simulink model "OR_10s_70l"  (R2023b)
(part 2 of 3)

      |     if contains(extractAfter(blocks{k,1}, '/'), 'Source')
      |         set_param(blocks{k}, 'BackgroundColor', '[0.929000, 0.490000, 0.439000]');
      |     end
      | end
      settings: NameChangeFcn=|
      | Component_Name = get_param(gcb, 'Name');
      | old_ID = get_param(gcb, 'Bus_ID');
      | 
      | pattern = '_\d+';
      | match = regexp(Component_Name, pattern, 'match');
      | 
      | if ~isempty(match)
      |     if ~isequal(old_ID, num2str(strtrim(extractAfter(Component_Name, '_'))))
      |         set_param(gcb, 'Bus_ID', num2str(strtrim(extractAfter(Component_Name, '_'))));
      |     end
      | else
      |     newName = [Component_Name '_' old_ID];
      |     set_param(gcb, 'Name', newName);
      | end
      | 
      | if ~isequal(old_ID, get_param(gcb, 'Bus_ID'))
      | 
      |     data = get_param(gcb, 'PortConnectivity');
      |     for i = 1:numel(data)
      |         sourceHandle = data(i,1).SrcBlock;
      |         if ~isempty(sourceHandle) && sourceHandle ~= -1
      |             sourceParams = get_param(sourceHandle, 'DialogParameters');
      |             fn = fieldnames(sourceParams);
      |             if contains(fn{2}, 'Source')
      |                 Bus_ID = get_param(gcb, 'Bus_ID');
      |                 set_param(sourceHandle, 'Source_ID', Bus_ID);
      |             end
      |         end
      |     end
      | 
      |     blocks = find_system(gcs, 'SearchDepth', 1, 'Type', 'Block');
      | 
      |     for k = 1:length(blocks)
      |         if contains(extractAfter(blocks{k,1}, '/'), 'Source')
      |             set_param(blocks{k}, 'BackgroundColor', '[0.929000, 0.490000, 0.439000]');
      |         end
      |     end
      | 
      | end
      settings: PreDeleteFcn=|
      | blocks = find_system(gcs, 'SearchDepth', 1, 'Type', 'Block');
      | 
      | for k = 1:length(blocks)
      |     if contains(extractAfter(blocks{k,1}, '/'), 'Source')
      |         set_param(blocks{k}, 'BackgroundColor', '[0.929000, 0.490000, 0.439000]');
      |     end
      | end
  Bus_60 : MATLAB Function  TreatAsAtomicUnit=on  mask{MyInitialization=0, Bus_ID=60, Fault_flag=1}
      mask prompts: Bus_ID "Bus ID"; Fault_flag "Fault flag"
      settings: CopyFcn=|
      | Component_Name = get_param(gcb, 'Name');
      | set_param(gcb, 'Bus_ID', num2str(strtrim(extractAfter(Component_Name, '_'))));
      | 
      | blocks = find_system(gcs, 'SearchDepth', 1, 'Type', 'Block');
      | 
      | for k = 1:length(blocks)
      |     if contains(extractAfter(blocks{k,1}, '/'), 'Source')
      |         set_param(blocks{k}, 'BackgroundColor', '[0.929000, 0.490000, 0.439000]');
      |     end
      | end
      settings: NameChangeFcn=|
      | Component_Name = get_param(gcb, 'Name');
      | old_ID = get_param(gcb, 'Bus_ID');
      | 
      | pattern = '_\d+';
      | match = regexp(Component_Name, pattern, 'match');
      | 
      | if ~isempty(match)
      |     if ~isequal(old_ID, num2str(strtrim(extractAfter(Component_Name, '_'))))
      |         set_param(gcb, 'Bus_ID', num2str(strtrim(extractAfter(Component_Name, '_'))));
      |     end
      | else
      |     newName = [Component_Name '_' old_ID];
      |     set_param(gcb, 'Name', newName);
      | end
      | 
      | if ~isequal(old_ID, get_param(gcb, 'Bus_ID'))
      | 
      |     data = get_param(gcb, 'PortConnectivity');
      |     for i = 1:numel(data)
      |         sourceHandle = data(i,1).SrcBlock;
      |         if ~isempty(sourceHandle) && sourceHandle ~= -1
      |             sourceParams = get_param(sourceHandle, 'DialogParameters');
      |             fn = fieldnames(sourceParams);
      |             if contains(fn{2}, 'Source')
      |                 Bus_ID = get_param(gcb, 'Bus_ID');
      |                 set_param(sourceHandle, 'Source_ID', Bus_ID);
      |             end
      |         end
      |     end
      | 
      |     blocks = find_system(gcs, 'SearchDepth', 1, 'Type', 'Block');
      | 
      |     for k = 1:length(blocks)
      |         if contains(extractAfter(blocks{k,1}, '/'), 'Source')
      |             set_param(blocks{k}, 'BackgroundColor', '[0.929000, 0.490000, 0.439000]');
      |         end
      |     end
      | 
      | end
      settings: PreDeleteFcn=|
      | blocks = find_system(gcs, 'SearchDepth', 1, 'Type', 'Block');
      | 
      | for k = 1:length(blocks)
      |     if contains(extractAfter(blocks{k,1}, '/'), 'Source')
      |         set_param(blocks{k}, 'BackgroundColor', '[0.929000, 0.490000, 0.439000]');
      |     end
      | end
  Bus_61 : MATLAB Function  TreatAsAtomicUnit=on  mask{MyInitialization=0, Bus_ID=61, Fault_flag=1}
      mask prompts: Bus_ID "Bus ID"; Fault_flag "Fault flag"
      settings: CopyFcn=|
      | Component_Name = get_param(gcb, 'Name');
      | set_param(gcb, 'Bus_ID', num2str(strtrim(extractAfter(Component_Name, '_'))));
      | 
      | blocks = find_system(gcs, 'SearchDepth', 1, 'Type', 'Block');
      | 
      | for k = 1:length(blocks)
      |     if contains(extractAfter(blocks{k,1}, '/'), 'Source')
      |         set_param(blocks{k}, 'BackgroundColor', '[0.929000, 0.490000, 0.439000]');
      |     end
      | end
      settings: NameChangeFcn=|
      | Component_Name = get_param(gcb, 'Name');
      | old_ID = get_param(gcb, 'Bus_ID');
      | 
      | pattern = '_\d+';
      | match = regexp(Component_Name, pattern, 'match');
      | 
      | if ~isempty(match)
      |     if ~isequal(old_ID, num2str(strtrim(extractAfter(Component_Name, '_'))))
      |         set_param(gcb, 'Bus_ID', num2str(strtrim(extractAfter(Component_Name, '_'))));
      |     end
      | else
      |     newName = [Component_Name '_' old_ID];
      |     set_param(gcb, 'Name', newName);
      | end
      | 
      | if ~isequal(old_ID, get_param(gcb, 'Bus_ID'))
      | 
      |     data = get_param(gcb, 'PortConnectivity');
      |     for i = 1:numel(data)
      |         sourceHandle = data(i,1).SrcBlock;
      |         if ~isempty(sourceHandle) && sourceHandle ~= -1
      |             sourceParams = get_param(sourceHandle, 'DialogParameters');
      |             fn = fieldnames(sourceParams);
      |             if contains(fn{2}, 'Source')
      |                 Bus_ID = get_param(gcb, 'Bus_ID');
      |                 set_param(sourceHandle, 'Source_ID', Bus_ID);
      |             end
      |         end
      |     end
      | 
      |     blocks = find_system(gcs, 'SearchDepth', 1, 'Type', 'Block');
      | 
      |     for k = 1:length(blocks)
      |         if contains(extractAfter(blocks{k,1}, '/'), 'Source')
      |             set_param(blocks{k}, 'BackgroundColor', '[0.929000, 0.490000, 0.439000]');
      |         end
      |     end
      | 
      | end
      settings: PreDeleteFcn=|
      | blocks = find_system(gcs, 'SearchDepth', 1, 'Type', 'Block');
      | 
      | for k = 1:length(blocks)
      |     if contains(extractAfter(blocks{k,1}, '/'), 'Source')
      |         set_param(blocks{k}, 'BackgroundColor', '[0.929000, 0.490000, 0.439000]');
      |     end
      | end
  Bus_62 : MATLAB Function  TreatAsAtomicUnit=on  mask{MyInitialization=0, Bus_ID=62, Fault_flag=1}
      mask prompts: Bus_ID "Bus ID"; Fault_flag "Fault flag"
      settings: CopyFcn=|
      | Component_Name = get_param(gcb, 'Name');
      | set_param(gcb, 'Bus_ID', num2str(strtrim(extractAfter(Component_Name, '_'))));
      | 
      | blocks = find_system(gcs, 'SearchDepth', 1, 'Type', 'Block');
      | 
      | for k = 1:length(blocks)
      |     if contains(extractAfter(blocks{k,1}, '/'), 'Source')
      |         set_param(blocks{k}, 'BackgroundColor', '[0.929000, 0.490000, 0.439000]');
      |     end
      | end
      settings: NameChangeFcn=|
      | Component_Name = get_param(gcb, 'Name');
      | old_ID = get_param(gcb, 'Bus_ID');
      | 
      | pattern = '_\d+';
      | match = regexp(Component_Name, pattern, 'match');
      | 
      | if ~isempty(match)
      |     if ~isequal(old_ID, num2str(strtrim(extractAfter(Component_Name, '_'))))
      |         set_param(gcb, 'Bus_ID', num2str(strtrim(extractAfter(Component_Name, '_'))));
      |     end
      | else
      |     newName = [Component_Name '_' old_ID];
      |     set_param(gcb, 'Name', newName);
      | end
      | 
      | if ~isequal(old_ID, get_param(gcb, 'Bus_ID'))
      | 
      |     data = get_param(gcb, 'PortConnectivity');
      |     for i = 1:numel(data)
      |         sourceHandle = data(i,1).SrcBlock;
      |         if ~isempty(sourceHandle) && sourceHandle ~= -1
      |             sourceParams = get_param(sourceHandle, 'DialogParameters');
      |             fn = fieldnames(sourceParams);
      |             if contains(fn{2}, 'Source')
      |                 Bus_ID = get_param(gcb, 'Bus_ID');
      |                 set_param(sourceHandle, 'Source_ID', Bus_ID);
      |             end
      |         end
      |     end
      | 
      |     blocks = find_system(gcs, 'SearchDepth', 1, 'Type', 'Block');
      | 
      |     for k = 1:length(blocks)
      |         if contains(extractAfter(blocks{k,1}, '/'), 'Source')
      |             set_param(blocks{k}, 'BackgroundColor', '[0.929000, 0.490000, 0.439000]');
      |         end
      |     end
      | 
      | end
      settings: PreDeleteFcn=|
      | blocks = find_system(gcs, 'SearchDepth', 1, 'Type', 'Block');
      | 
      | for k = 1:length(blocks)
      |     if contains(extractAfter(blocks{k,1}, '/'), 'Source')
      |         set_param(blocks{k}, 'BackgroundColor', '[0.929000, 0.490000, 0.439000]');
      |     end
      | end
  Bus_63 : MATLAB Function  TreatAsAtomicUnit=on  mask{MyInitialization=0, Bus_ID=63, Fault_flag=1}
      mask prompts: Bus_ID "Bus ID"; Fault_flag "Fault flag"
      settings: CopyFcn=|
      | Component_Name = get_param(gcb, 'Name');
      | set_param(gcb, 'Bus_ID', num2str(strtrim(extractAfter(Component_Name, '_'))));
      | 
      | blocks = find_system(gcs, 'SearchDepth', 1, 'Type', 'Block');
      | 
      | for k = 1:length(blocks)
      |     if contains(extractAfter(blocks{k,1}, '/'), 'Source')
      |         set_param(blocks{k}, 'BackgroundColor', '[0.929000, 0.490000, 0.439000]');
      |     end
      | end
      settings: NameChangeFcn=|
      | Component_Name = get_param(gcb, 'Name');
      | old_ID = get_param(gcb, 'Bus_ID');
      | 
      | pattern = '_\d+';
      | match = regexp(Component_Name, pattern, 'match');
      | 
      | if ~isempty(match)
      |     if ~isequal(old_ID, num2str(strtrim(extractAfter(Component_Name, '_'))))
      |         set_param(gcb, 'Bus_ID', num2str(strtrim(extractAfter(Component_Name, '_'))));
      |     end
      | else
      |     newName = [Component_Name '_' old_ID];
      |     set_param(gcb, 'Name', newName);
      | end
      | 
      | if ~isequal(old_ID, get_param(gcb, 'Bus_ID'))
      | 
      |     data = get_param(gcb, 'PortConnectivity');
      |     for i = 1:numel(data)
      |         sourceHandle = data(i,1).SrcBlock;
      |         if ~isempty(sourceHandle) && sourceHandle ~= -1
      |             sourceParams = get_param(sourceHandle, 'DialogParameters');
      |             fn = fieldnames(sourceParams);
      |             if contains(fn{2}, 'Source')
      |                 Bus_ID = get_param(gcb, 'Bus_ID');
      |                 set_param(sourceHandle, 'Source_ID', Bus_ID);
      |             end
      |         end
      |     end
      | 
      |     blocks = find_system(gcs, 'SearchDepth', 1, 'Type', 'Block');
      | 
      |     for k = 1:length(blocks)
      |         if contains(extractAfter(blocks{k,1}, '/'), 'Source')
      |             set_param(blocks{k}, 'BackgroundColor', '[0.929000, 0.490000, 0.439000]');
      |         end
      |     end
      | 
      | end
      settings: PreDeleteFcn=|
      | blocks = find_system(gcs, 'SearchDepth', 1, 'Type', 'Block');
      | 
      | for k = 1:length(blocks)
      |     if contains(extractAfter(blocks{k,1}, '/'), 'Source')
      |         set_param(blocks{k}, 'BackgroundColor', '[0.929000, 0.490000, 0.439000]');
      |     end
      | end
  Bus_64 : MATLAB Function  TreatAsAtomicUnit=on  mask{MyInitialization=0, Bus_ID=64, Fault_flag=1}
      mask prompts: Bus_ID "Bus ID"; Fault_flag "Fault flag"
      settings: CopyFcn=|
      | Component_Name = get_param(gcb, 'Name');
      | set_param(gcb, 'Bus_ID', num2str(strtrim(extractAfter(Component_Name, '_'))));
      | 
      | blocks = find_system(gcs, 'SearchDepth', 1, 'Type', 'Block');
      | 
      | for k = 1:length(blocks)
      |     if contains(extractAfter(blocks{k,1}, '/'), 'Source')
      |         set_param(blocks{k}, 'BackgroundColor', '[0.929000, 0.490000, 0.439000]');
      |     end
      | end
      settings: NameChangeFcn=|
      | Component_Name = get_param(gcb, 'Name');
      | old_ID = get_param(gcb, 'Bus_ID');
      | 
      | pattern = '_\d+';
      | match = regexp(Component_Name, pattern, 'match');
      | 
      | if ~isempty(match)
      |     if ~isequal(old_ID, num2str(strtrim(extractAfter(Component_Name, '_'))))
      |         set_param(gcb, 'Bus_ID', num2str(strtrim(extractAfter(Component_Name, '_'))));
      |     end
      | else
      |     newName = [Component_Name '_' old_ID];
      |     set_param(gcb, 'Name', newName);
      | end
      | 
      | if ~isequal(old_ID, get_param(gcb, 'Bus_ID'))
      | 
      |     data = get_param(gcb, 'PortConnectivity');
      |     for i = 1:numel(data)
      |         sourceHandle = data(i,1).SrcBlock;
      |         if ~isempty(sourceHandle) && sourceHandle ~= -1
      |             sourceParams = get_param(sourceHandle, 'DialogParameters');
      |             fn = fieldnames(sourceParams);
      |             if contains(fn{2}, 'Source')
      |                 Bus_ID = get_param(gcb, 'Bus_ID');
      |                 set_param(sourceHandle, 'Source_ID', Bus_ID);
      |             end
      |         end
      |     end
      | 
      |     blocks = find_system(gcs, 'SearchDepth', 1, 'Type', 'Block');
      | 
      |     for k = 1:length(blocks)
      |         if contains(extractAfter(blocks{k,1}, '/'), 'Source')
      |             set_param(blocks{k}, 'BackgroundColor', '[0.929000, 0.490000, 0.439000]');
      |         end
      |     end
      | 
      | end
      settings: PreDeleteFcn=|
      | blocks = find_system(gcs, 'SearchDepth', 1, 'Type', 'Block');
      | 
      | for k = 1:length(blocks)
      |     if contains(extractAfter(blocks{k,1}, '/'), 'Source')
      |         set_param(blocks{k}, 'BackgroundColor', '[0.929000, 0.490000, 0.439000]');
      |     end
      | end
  Bus_65 : MATLAB Function  TreatAsAtomicUnit=on  mask{MyInitialization=0, Bus_ID=65, Fault_flag=1}
      mask prompts: Bus_ID "Bus ID"; Fault_flag "Fault flag"
      settings: CopyFcn=|
      | Component_Name = get_param(gcb, 'Name');
      | set_param(gcb, 'Bus_ID', num2str(strtrim(extractAfter(Component_Name, '_'))));
      | 
      | blocks = find_system(gcs, 'SearchDepth', 1, 'Type', 'Block');
      | 
      | for k = 1:length(blocks)
      |     if contains(extractAfter(blocks{k,1}, '/'), 'Source')
      |         set_param(blocks{k}, 'BackgroundColor', '[0.929000, 0.490000, 0.439000]');
      |     end
      | end
      settings: NameChangeFcn=|
      | Component_Name = get_param(gcb, 'Name');
      | old_ID = get_param(gcb, 'Bus_ID');
      | 
      | pattern = '_\d+';
      | match = regexp(Component_Name, pattern, 'match');
      | 
      | if ~isempty(match)
      |     if ~isequal(old_ID, num2str(strtrim(extractAfter(Component_Name, '_'))))
      |         set_param(gcb, 'Bus_ID', num2str(strtrim(extractAfter(Component_Name, '_'))));
      |     end
      | else
      |     newName = [Component_Name '_' old_ID];
      |     set_param(gcb, 'Name', newName);
      | end
      | 
      | if ~isequal(old_ID, get_param(gcb, 'Bus_ID'))
      | 
      |     data = get_param(gcb, 'PortConnectivity');
      |     for i = 1:numel(data)
      |         sourceHandle = data(i,1).SrcBlock;
      |         if ~isempty(sourceHandle) && sourceHandle ~= -1
      |             sourceParams = get_param(sourceHandle, 'DialogParameters');
      |             fn = fieldnames(sourceParams);
      |             if contains(fn{2}, 'Source')
      |                 Bus_ID = get_param(gcb, 'Bus_ID');
      |                 set_param(sourceHandle, 'Source_ID', Bus_ID);
      |             end
      |         end
      |     end
      | 
      |     blocks = find_system(gcs, 'SearchDepth', 1, 'Type', 'Block');
      | 
      |     for k = 1:length(blocks)
      |         if contains(extractAfter(blocks{k,1}, '/'), 'Source')
      |             set_param(blocks{k}, 'BackgroundColor', '[0.929000, 0.490000, 0.439000]');
      |         end
      |     end
      | 
      | end
      settings: PreDeleteFcn=|
      | blocks = find_system(gcs, 'SearchDepth', 1, 'Type', 'Block');
      | 
      | for k = 1:length(blocks)
      |     if contains(extractAfter(blocks{k,1}, '/'), 'Source')
      |         set_param(blocks{k}, 'BackgroundColor', '[0.929000, 0.490000, 0.439000]');
      |     end
      | end
  Bus_7 : MATLAB Function  TreatAsAtomicUnit=on  mask{MyInitialization=0, Bus_ID=7, Fault_flag=1}
      mask prompts: Bus_ID "Bus ID"; Fault_flag "Fault flag"
      settings: CopyFcn=|
      | Component_Name = get_param(gcb, 'Name');
      | set_param(gcb, 'Bus_ID', num2str(strtrim(extractAfter(Component_Name, '_'))));
      | 
      | blocks = find_system(gcs, 'SearchDepth', 1, 'Type', 'Block');
      | 
      | for k = 1:length(blocks)
      |     if contains(extractAfter(blocks{k,1}, '/'), 'Source')
      |         set_param(blocks{k}, 'BackgroundColor', '[0.929000, 0.490000, 0.439000]');
      |     end
      | end
      settings: NameChangeFcn=|
      | Component_Name = get_param(gcb, 'Name');
      | old_ID = get_param(gcb, 'Bus_ID');
      | 
      | pattern = '_\d+';
      | match = regexp(Component_Name, pattern, 'match');
      | 
      | if ~isempty(match)
      |     if ~isequal(old_ID, num2str(strtrim(extractAfter(Component_Name, '_'))))
      |         set_param(gcb, 'Bus_ID', num2str(strtrim(extractAfter(Component_Name, '_'))));
      |     end
      | else
      |     newName = [Component_Name '_' old_ID];
      |     set_param(gcb, 'Name', newName);
      | end
      | 
      | if ~isequal(old_ID, get_param(gcb, 'Bus_ID'))
      | 
      |     data = get_param(gcb, 'PortConnectivity');
      |     for i = 1:numel(data)
      |         sourceHandle = data(i,1).SrcBlock;
      |         if ~isempty(sourceHandle) && sourceHandle ~= -1
      |             sourceParams = get_param(sourceHandle, 'DialogParameters');
      |             fn = fieldnames(sourceParams);
      |             if contains(fn{2}, 'Source')
      |                 Bus_ID = get_param(gcb, 'Bus_ID');
      |                 set_param(sourceHandle, 'Source_ID', Bus_ID);
      |             end
      |         end
      |     end
      | 
      |     blocks = find_system(gcs, 'SearchDepth', 1, 'Type', 'Block');
      | 
      |     for k = 1:length(blocks)
      |         if contains(extractAfter(blocks{k,1}, '/'), 'Source')
      |             set_param(blocks{k}, 'BackgroundColor', '[0.929000, 0.490000, 0.439000]');
      |         end
      |     end
      | 
      | end
      settings: PreDeleteFcn=|
      | blocks = find_system(gcs, 'SearchDepth', 1, 'Type', 'Block');
      | 
      | for k = 1:length(blocks)
      |     if contains(extractAfter(blocks{k,1}, '/'), 'Source')
      |         set_param(blocks{k}, 'BackgroundColor', '[0.929000, 0.490000, 0.439000]');
      |     end
      | end
  Bus_8 : MATLAB Function  TreatAsAtomicUnit=on  mask{MyInitialization=0, Bus_ID=8, Fault_flag=0}
      mask prompts: Bus_ID "Bus ID"; Fault_flag "Fault flag"
      settings: CopyFcn=|
      | Component_Name = get_param(gcb, 'Name');
      | set_param(gcb, 'Bus_ID', num2str(strtrim(extractAfter(Component_Name, '_'))));
      | 
      | blocks = find_system(gcs, 'SearchDepth', 1, 'Type', 'Block');
      | 
      | for k = 1:length(blocks)
      |     if contains(extractAfter(blocks{k,1}, '/'), 'Source')
      |         set_param(blocks{k}, 'BackgroundColor', '[0.929000, 0.490000, 0.439000]');
      |     end
      | end
      settings: NameChangeFcn=|
      | Component_Name = get_param(gcb, 'Name');
      | old_ID = get_param(gcb, 'Bus_ID');
      | 
      | pattern = '_\d+';
      | match = regexp(Component_Name, pattern, 'match');
      | 
      | if ~isempty(match)
      |     if ~isequal(old_ID, num2str(strtrim(extractAfter(Component_Name, '_'))))
      |         set_param(gcb, 'Bus_ID', num2str(strtrim(extractAfter(Component_Name, '_'))));
      |     end
      | else
      |     newName = [Component_Name '_' old_ID];
      |     set_param(gcb, 'Name', newName);
      | end
      | 
      | if ~isequal(old_ID, get_param(gcb, 'Bus_ID'))
      | 
      |     data = get_param(gcb, 'PortConnectivity');
      |     for i = 1:numel(data)
      |         sourceHandle = data(i,1).SrcBlock;
      |         if ~isempty(sourceHandle) && sourceHandle ~= -1
      |             sourceParams = get_param(sourceHandle, 'DialogParameters');
      |             fn = fieldnames(sourceParams);
      |             if contains(fn{2}, 'Source')
      |                 Bus_ID = get_param(gcb, 'Bus_ID');
      |                 set_param(sourceHandle, 'Source_ID', Bus_ID);
      |             end
      |         end
      |     end
      | 
      |     blocks = find_system(gcs, 'SearchDepth', 1, 'Type', 'Block');
      | 
      |     for k = 1:length(blocks)
      |         if contains(extractAfter(blocks{k,1}, '/'), 'Source')
      |             set_param(blocks{k}, 'BackgroundColor', '[0.929000, 0.490000, 0.439000]');
      |         end
      |     end
      | 
      | end
      settings: PreDeleteFcn=|
      | blocks = find_system(gcs, 'SearchDepth', 1, 'Type', 'Block');
      | 
      | for k = 1:length(blocks)
      |     if contains(extractAfter(blocks{k,1}, '/'), 'Source')
      |         set_param(blocks{k}, 'BackgroundColor', '[0.929000, 0.490000, 0.439000]');
      |     end
      | end
  Bus_9 : MATLAB Function  TreatAsAtomicUnit=on  mask{MyInitialization=0, Bus_ID=9, Fault_flag=1}
      mask prompts: Bus_ID "Bus ID"; Fault_flag "Fault flag"
      settings: CopyFcn=|
      | Component_Name = get_param(gcb, 'Name');
      | set_param(gcb, 'Bus_ID', num2str(strtrim(extractAfter(Component_Name, '_'))));
      | 
      | blocks = find_system(gcs, 'SearchDepth', 1, 'Type', 'Block');
      | 
      | for k = 1:length(blocks)
      |     if contains(extractAfter(blocks{k,1}, '/'), 'Source')
      |         set_param(blocks{k}, 'BackgroundColor', '[0.929000, 0.490000, 0.439000]');
      |     end
      | end
      settings: NameChangeFcn=|
      | Component_Name = get_param(gcb, 'Name');
      | old_ID = get_param(gcb, 'Bus_ID');
      | 
      | pattern = '_\d+';
      | match = regexp(Component_Name, pattern, 'match');
      | 
      | if ~isempty(match)
      |     if ~isequal(old_ID, num2str(strtrim(extractAfter(Component_Name, '_'))))
      |         set_param(gcb, 'Bus_ID', num2str(strtrim(extractAfter(Component_Name, '_'))));
      |     end
      | else
      |     newName = [Component_Name '_' old_ID];
      |     set_param(gcb, 'Name', newName);
      | end
      | 
      | if ~isequal(old_ID, get_param(gcb, 'Bus_ID'))
      | 
      |     data = get_param(gcb, 'PortConnectivity');
      |     for i = 1:numel(data)
      |         sourceHandle = data(i,1).SrcBlock;
      |         if ~isempty(sourceHandle) && sourceHandle ~= -1
      |             sourceParams = get_param(sourceHandle, 'DialogParameters');
      |             fn = fieldnames(sourceParams);
      |             if contains(fn{2}, 'Source')
      |                 Bus_ID = get_param(gcb, 'Bus_ID');
      |                 set_param(sourceHandle, 'Source_ID', Bus_ID);
      |             end
      |         end
      |     end
      | 
      |     blocks = find_system(gcs, 'SearchDepth', 1, 'Type', 'Block');
      | 
      |     for k = 1:length(blocks)
      |         if contains(extractAfter(blocks{k,1}, '/'), 'Source')
      |             set_param(blocks{k}, 'BackgroundColor', '[0.929000, 0.490000, 0.439000]');
      |         end
      |     end
      | 
      | end
      settings: PreDeleteFcn=|
      | blocks = find_system(gcs, 'SearchDepth', 1, 'Type', 'Block');
      | 
      | for k = 1:length(blocks)
      |     if contains(extractAfter(blocks{k,1}, '/'), 'Source')
      |         set_param(blocks{k}, 'BackgroundColor', '[0.929000, 0.490000, 0.439000]');
      |     end
      | end
  CB_1 : ABB_UPPAAL_Library/CB_1  MyInitialization=0  CB_ID=1  Sel_Type=3  m=3  i1=900  t1=180  i2_flag=off  i2=null  t2=null  i3_flag=off  i3=null  t3=null  i7=1800  t7FW=8  t7BW=8  tselFW=1  tselBW=1  Actors={ '3', '1', '1' }
      settings: SourceProductName=ABB UPPAAL Library
  CB_10 : ABB_UPPAAL_Library/CB_1  MyInitialization=0  CB_ID=10  Sel_Type=1  m=3  i1=90  t1=160  i2_flag=on  i2=180  t2=6  i3_flag=off  i3=null  t3=null  i7=null  t7FW=null  t7BW=null  tselFW=null  tselBW=null  Actors={}
      settings: SourceProductName=ABB UPPAAL Library
  CB_11 : ABB_UPPAAL_Library/CB_1  MyInitialization=0  CB_ID=11  Sel_Type=1  m=3  i1=30  t1=100  i2_flag=on  i2=60  t2=2  i3_flag=off  i3=null  t3=null  i7=null  t7FW=null  t7BW=null  tselFW=null  tselBW=null  Actors={}
      settings: SourceProductName=ABB UPPAAL Library
  CB_12 : ABB_UPPAAL_Library/CB_1  MyInitialization=0  CB_ID=12  Sel_Type=1  m=3  i1=60  t1=120  i2_flag=on  i2=120  t2=4  i3_flag=off  i3=null  t3=null  i7=null  t7FW=null  t7BW=null  tselFW=null  tselBW=null  Actors={}
      settings: SourceProductName=ABB UPPAAL Library
  CB_13 : ABB_UPPAAL_Library/CB_1  MyInitialization=0  CB_ID=13  Sel_Type=1  m=3  i1=30  t1=100  i2_flag=on  i2=60  t2=2  i3_flag=off  i3=null  t3=null  i7=null  t7FW=null  t7BW=null  tselFW=null  tselBW=null  Actors={}
      settings: SourceProductName=ABB UPPAAL Library
  CB_14 : ABB_UPPAAL_Library/CB_1  MyInitialization=0  CB_ID=14  Sel_Type=1  m=3  i1=30  t1=100  i2_flag=on  i2=60  t2=2  i3_flag=off  i3=null  t3=null  i7=null  t7FW=null  t7BW=null  tselFW=null  tselBW=null  Actors={}
      settings: SourceProductName=ABB UPPAAL Library
  CB_15 : ABB_UPPAAL_Library/CB_1  MyInitialization=0  CB_ID=15  Sel_Type=3  m=3  i1=720  t1=170  i2_flag=off  i2=null  t2=null  i3_flag=off  i3=null  t3=null  i7=1440  t7FW=7  t7BW=7  tselFW=1  tselBW=1  Actors={ '8', '0', '0'; '9', '0', '0'; '10', '1', '0'; '16', '0', '1'; '17', '1', '1'; '22', '1', '1' }
      settings: SourceProductName=ABB UPPAAL Library
  CB_16 : ABB_UPPAAL_Library/CB_1  MyInitialization=0  CB_ID=16  Sel_Type=3  m=3  i1=900  t1=180  i2_flag=off  i2=null  t2=null  i3_flag=off  i3=null  t3=null  i7=1800  t7FW=8  t7BW=8  tselFW=1  tselBW=1  Actors={ '15', '0', '1'; '17', '1', '1'; '22', '1', '1' }
      settings: SourceProductName=ABB UPPAAL Library
  CB_17 : ABB_UPPAAL_Library/CB_1  MyInitialization=0  CB_ID=17  Sel_Type=1  m=3  i1=90  t1=160  i2_flag=on  i2=180  t2=6  i3_flag=off  i3=null  t3=null  i7=null  t7FW=null  t7BW=null  tselFW=null  tselBW=null  Actors={}
      settings: SourceProductName=ABB UPPAAL Library
  CB_18 : ABB_UPPAAL_Library/CB_1  MyInitialization=0  CB_ID=18  Sel_Type=1  m=3  i1=30  t1=100  i2_flag=on  i2=60  t2=2  i3_flag=off  i3=null  t3=null  i7=null  t7FW=null  t7BW=null  tselFW=null  tselBW=null  Actors={}
      settings: SourceProductName=ABB UPPAAL Library
  CB_19 : ABB_UPPAAL_Library/CB_1  MyInitialization=0  CB_ID=19  Sel_Type=1  m=3  i1=30  t1=100  i2_flag=on  i2=60  t2=2  i3_flag=off  i3=null  t3=null  i7=null  t7FW=null  t7BW=null  tselFW=null  tselBW=null  Actors={}
      settings: SourceProductName=ABB UPPAAL Library
  CB_2 : ABB_UPPAAL_Library/CB_1  MyInitialization=0  CB_ID=2  Sel_Type=3  m=3  i1=900  t1=180  i2_flag=off  i2=null  t2=null  i3_flag=off  i3=null  t3=null  i7=1800  t7FW=8  t7BW=8  tselFW=1  tselBW=1  Actors={ '3', '0', '1'; '4', '1', '1'; '9', '1', '1' }
      settings: SourceProductName=ABB UPPAAL Library
  CB_20 : ABB_UPPAAL_Library/CB_1  MyInitialization=0  CB_ID=20  Sel_Type=1  m=3  i1=30  t1=100  i2_flag=on  i2=60  t2=2  i3_flag=off  i3=null  t3=null  i7=null  t7FW=null  t7BW=null  tselFW=null  tselBW=null  Actors={}
      settings: SourceProductName=ABB UPPAAL Library
  CB_21 : ABB_UPPAAL_Library/CB_1  MyInitialization=0  CB_ID=21  Sel_Type=3  m=3  i1=900  t1=180  i2_flag=off  i2=null  t2=null  i3_flag=off  i3=null  t3=null  i7=1800  t7FW=8  t7BW=8  tselFW=1  tselBW=1  Actors={ '22', '0', '1'; '30', '1', '1'; '31', '1', '1' }
      settings: SourceProductName=ABB UPPAAL Library
  CB_22 : ABB_UPPAAL_Library/CB_1  MyInitialization=0  CB_ID=22  Sel_Type=3  m=3  i1=630  t1=170  i2_flag=off  i2=null  t2=null  i3_flag=off  i3=null  t3=null  i7=1260  t7FW=7  t7BW=7  tselFW=1  tselBW=1  Actors={ '15', '0', '0'; '16', '0', '0'; '17', '1', '0'; '21', '0', '1'; '30', '1', '1'; '31', '1', '1' }
      settings: SourceProductName=ABB UPPAAL Library
  CB_23 : ABB_UPPAAL_Library/CB_1  MyInitialization=0  CB_ID=23  Sel_Type=1  m=3  i1=90  t1=160  i2_flag=on  i2=180  t2=6  i3_flag=off  i3=null  t3=null  i7=null  t7FW=null  t7BW=null  tselFW=null  tselBW=null  Actors={}
      settings: SourceProductName=ABB UPPAAL Library
  CB_24 : ABB_UPPAAL_Library/CB_1  MyInitialization=0  CB_ID=24  Sel_Type=1  m=3  i1=30  t1=100  i2_flag=on  i2=60  t2=2  i3_flag=off  i3=null  t3=null  i7=null  t7FW=null  t7BW=null  tselFW=null  tselBW=null  Actors={}
      settings: SourceProductName=ABB UPPAAL Library
  CB_25 : ABB_UPPAAL_Library/CB_1  MyInitialization=0  CB_ID=25  Sel_Type=1  m=3  i1=60  t1=120  i2_flag=on  i2=120  t2=4  i3_flag=off  i3=null  t3=null  i7=null  t7FW=null  t7BW=null  tselFW=null  tselBW=null  Actors={}
      settings: SourceProductName=ABB UPPAAL Library
  CB_26 : ABB_UPPAAL_Library/CB_1  MyInitialization=0  CB_ID=26  Sel_Type=1  m=3  i1=30  t1=100  i2_flag=on  i2=60  t2=2  i3_flag=off  i3=null  t3=null  i7=null  t7FW=null  t7BW=null  tselFW=null  tselBW=null  Actors={}
      settings: SourceProductName=ABB UPPAAL Library
  CB_27 : ABB_UPPAAL_Library/CB_1  MyInitialization=0  CB_ID=27  Sel_Type=1  m=3  i1=30  t1=100  i2_flag=on  i2=60  t2=2  i3_flag=off  i3=null  t3=null  i7=null  t7FW=null  t7BW=null  tselFW=null  tselBW=null  Actors={}
      settings: SourceProductName=ABB UPPAAL Library
  CB_28 : ABB_UPPAAL_Library/CB_1  MyInitialization=0  CB_ID=28  Sel_Type=3  m=3  i1=310  t1=170  i2_flag=off  i2=null  t2=null  i3_flag=off  i3=null  t3=null  i7=620  t7FW=7  t7BW=7  tselFW=1  tselBW=1  Actors={ '23', '1', '0'; '29', '0', '0'; '30', '0', '0'; '32', '1', '1'; '37', '1', '1'; '38', '0', '1' }
      settings: SourceProductName=ABB UPPAAL Library
  CB_29 : ABB_UPPAAL_Library/CB_1  MyInitialization=0  CB_ID=29  Sel_Type=3  m=3  i1=900  t1=180  i2_flag=off  i2=null  t2=null  i3_flag=off  i3=null  t3=null  i7=1800  t7FW=8  t7BW=8  tselFW=1  tselBW=1  Actors={ '23', '1', '1'; '28', '1', '1'; '30', '0', '1' }
      settings: SourceProductName=ABB UPPAAL Library
  CB_3 : ABB_UPPAAL_Library/CB_1  MyInitialization=0  CB_ID=3  Sel_Type=3  m=3  i1=900  t1=170  i2_flag=off  i2=null  t2=null  i3_flag=off  i3=null  t3=null  i7=1800  t7FW=7  t7BW=7  tselFW=1  tselBW=1  Actors={ '1', '0', '0'; '2', '0', '1'; '4', '1', '1'; '9', '1', '1' }
      settings: SourceProductName=ABB UPPAAL Library
  CB_30 : ABB_UPPAAL_Library/CB_1  MyInitialization=0  CB_ID=30  Sel_Type=3  m=3  i1=600  t1=170  i2_flag=off  i2=null  t2=null  i3_flag=off  i3=null  t3=null  i7=1200  t7FW=7  t7BW=7  tselFW=1  tselBW=1  Actors={ '21', '0', '0'; '22', '0', '0'; '23', '1', '1'; '28', '1', '1'; '29', '0', '1'; '31', '1', '0' }
      settings: SourceProductName=ABB UPPAAL Library
  CB_31 : ABB_UPPAAL_Library/CB_1  MyInitialization=0  CB_ID=31  Sel_Type=1  m=3  i1=30  t1=100  i2_flag=on  i2=60  t2=2  i3_flag=off  i3=null  t3=null  i7=null  t7FW=null  t7BW=null  tselFW=null  tselBW=null  Actors={}
      settings: SourceProductName=ABB UPPAAL Library
  CB_32 : ABB_UPPAAL_Library/CB_1  MyInitialization=0  CB_ID=32  Sel_Type=1  m=3  i1=90  t1=160  i2_flag=on  i2=180  t2=6  i3_flag=off  i3=null  t3=null  i7=null  t7FW=null  t7BW=null  tselFW=null  tselBW=null  Actors={}
      settings: SourceProductName=ABB UPPAAL Library
  CB_33 : ABB_UPPAAL_Library/CB_1  MyInitialization=0  CB_ID=33  Sel_Type=1  m=3  i1=30  t1=100  i2_flag=on  i2=60  t2=2  i3_flag=off  i3=null  t3=null  i7=null  t7FW=null  t7BW=null  tselFW=null  tselBW=null  Actors={}
      settings: SourceProductName=ABB UPPAAL Library
  CB_34 : ABB_UPPAAL_Library/CB_1  MyInitialization=0  CB_ID=34  Sel_Type=1  m=3  i1=60  t1=120  i2_flag=on  i2=120  t2=4  i3_flag=off  i3=null  t3=null  i7=null  t7FW=null  t7BW=null  tselFW=null  tselBW=null  Actors={}
      settings: SourceProductName=ABB UPPAAL Library
  CB_35 : ABB_UPPAAL_Library/CB_1  MyInitialization=0  CB_ID=35  Sel_Type=1  m=3  i1=30  t1=100  i2_flag=on  i2=60  t2=2  i3_flag=off  i3=null  t3=null  i7=null  t7FW=null  t7BW=null  tselFW=null  tselBW=null  Actors={}
      settings: SourceProductName=ABB UPPAAL Library
  CB_36 : ABB_UPPAAL_Library/CB_1  MyInitialization=0  CB_ID=36  Sel_Type=1  m=3  i1=30  t1=100  i2_flag=on  i2=60  t2=2  i3_flag=off  i3=null  t3=null  i7=null  t7FW=null  t7BW=null  tselFW=null  tselBW=null  Actors={}
      settings: SourceProductName=ABB UPPAAL Library
  CB_37 : ABB_UPPAAL_Library/CB_1  MyInitialization=0  CB_ID=37  Sel_Type=3  m=3  i1=480  t1=170  i2_flag=off  i2=null  t2=null  i3_flag=off  i3=null  t3=null  i7=960  t7FW=7  t7BW=7  tselFW=1  tselBW=1  Actors={ '28', '0', '0'; '32', '1', '0'; '38', '0', '0'; '39', '1', '1'; '44', '1', '1'; '45', '0', '1' }
      settings: SourceProductName=ABB UPPAAL Library
  CB_38 : ABB_UPPAAL_Library/CB_1  MyInitialization=0  CB_ID=38  Sel_Type=3  m=3  i1=900  t1=180  i2_flag=off  i2=null  t2=null  i3_flag=off  i3=null  t3=null  i7=1800  t7FW=8  t7BW=8  tselFW=1  tselBW=1  Actors={ '28', '0', '1'; '32', '1', '1'; '37', '1', '1' }
      settings: SourceProductName=ABB UPPAAL Library
  CB_39 : ABB_UPPAAL_Library/CB_1  MyInitialization=0  CB_ID=39  Sel_Type=1  m=3  i1=90  t1=160  i2_flag=on  i2=180  t2=6  i3_flag=off  i3=null  t3=null  i7=null  t7FW=null  t7BW=null  tselFW=null  tselBW=null  Actors={}
      settings: SourceProductName=ABB UPPAAL Library
  CB_4 : ABB_UPPAAL_Library/CB_1  MyInitialization=0  CB_ID=4  Sel_Type=1  m=3  i1=90  t1=120  i2_flag=on  i2=180  t2=4  i3_flag=off  i3=null  t3=null  i7=null  t7FW=null  t7BW=null  tselFW=null  tselBW=null  Actors={}
      settings: SourceProductName=ABB UPPAAL Library
  CB_40 : ABB_UPPAAL_Library/CB_1  MyInitialization=0  CB_ID=40  Sel_Type=1  m=3  i1=30  t1=100  i2_flag=on  i2=60  t2=2  i3_flag=off  i3=null  t3=null  i7=null  t7FW=null  t7BW=null  tselFW=null  tselBW=null  Actors={}
      settings: SourceProductName=ABB UPPAAL Library
  CB_41 : ABB_UPPAAL_Library/CB_1  MyInitialization=0  CB_ID=41  Sel_Type=1  m=3  i1=60  t1=120  i2_flag=on  i2=120  t2=4  i3_flag=off  i3=null  t3=null  i7=null  t7FW=null  t7BW=null  tselFW=null  tselBW=null  Actors={}
      settings: SourceProductName=ABB UPPAAL Library
  CB_42 : ABB_UPPAAL_Library/CB_1  MyInitialization=0  CB_ID=42  Sel_Type=1  m=3  i1=30  t1=100  i2_flag=on  i2=60  t2=2  i3_flag=off  i3=null  t3=null  i7=null  t7FW=null  t7BW=null  tselFW=null  tselBW=null  Actors={}
      settings: SourceProductName=ABB UPPAAL Library
  CB_43 : ABB_UPPAAL_Library/CB_1  MyInitialization=0  CB_ID=43  Sel_Type=1  m=3  i1=30  t1=100  i2_flag=on  i2=60  t2=2  i3_flag=off  i3=null  t3=null  i7=null  t7FW=null  t7BW=null  tselFW=null  tselBW=null  Actors={}
      settings: SourceProductName=ABB UPPAAL Library
  CB_44 : ABB_UPPAAL_Library/CB_1  MyInitialization=0  CB_ID=44  Sel_Type=3  m=3  i1=570  t1=170  i2_flag=off  i2=null  t2=null  i3_flag=off  i3=null  t3=null  i7=1140  t7FW=7  t7BW=7  tselFW=1  tselBW=1  Actors={ '37', '0', '0'; '39', '1', '0'; '45', '0', '0'; '46', '1', '1'; '51', '1', '1'; '52', '0', '1' }
      settings: SourceProductName=ABB UPPAAL Library
  CB_45 : ABB_UPPAAL_Library/CB_1  MyInitialization=0  CB_ID=45  Sel_Type=3  m=3  i1=900  t1=180  i2_flag=off  i2=null  t2=null  i3_flag=off  i3=null  t3=null  i7=1800  t7FW=8  t7BW=8  tselFW=1  tselBW=1  Actors={ '37', '0', '1'; '39', '1', '1'; '44', '1', '1' }
      settings: SourceProductName=ABB UPPAAL Library
  CB_46 : ABB_UPPAAL_Library/CB_1  MyInitialization=0  CB_ID=46  Sel_Type=1  m=3  i1=90  t1=160  i2_flag=on  i2=180  t2=6  i3_flag=off  i3=null  t3=null  i7=null  t7FW=null  t7BW=null  tselFW=null  tselBW=null  Actors={}
      settings: SourceProductName=ABB UPPAAL Library
  CB_47 : ABB_UPPAAL_Library/CB_1  MyInitialization=0  CB_ID=47  Sel_Type=1  m=3  i1=30  t1=100  i2_flag=on  i2=60  t2=2  i3_flag=off  i3=null  t3=null  i7=null  t7FW=null  t7BW=null  tselFW=null  tselBW=null  Actors={}
      settings: SourceProductName=ABB UPPAAL Library
  CB_48 : ABB_UPPAAL_Library/CB_1  MyInitialization=0  CB_ID=48  Sel_Type=1  m=3  i1=30  t1=100  i2_flag=on  i2=60  t2=2  i3_flag=off  i3=null  t3=null  i7=null  t7FW=null  t7BW=null  tselFW=null  tselBW=null  Actors={}
      settings: SourceProductName=ABB UPPAAL Library
  CB_49 : ABB_UPPAAL_Library/CB_1  MyInitialization=0  CB_ID=49  Sel_Type=1  m=3  i1=30  t1=100  i2_flag=on  i2=60  t2=2  i3_flag=off  i3=null  t3=null  i7=null  t7FW=null  t7BW=null  tselFW=null  tselBW=null  Actors={}
      settings: SourceProductName=ABB UPPAAL Library
  CB_5 : ABB_UPPAAL_Library/CB_1  MyInitialization=0  CB_ID=5  Sel_Type=1  m=3  i1=30  t1=100  i2_flag=on  i2=60  t2=2  i3_flag=off  i3=null  t3=null  i7=null  t7FW=null  t7BW=null  tselFW=null  tselBW=null  Actors={}
      settings: SourceProductName=ABB UPPAAL Library
  CB_50 : ABB_UPPAAL_Library/CB_1  MyInitialization=0  CB_ID=50  Sel_Type=1  m=null  i1=null  t1=null  i2_flag=off  i2=null  t2=null  i3_flag=off  i3=null  t3=null  i7=null  t7FW=null  t7BW=null  tselFW=null  tselBW=null  Actors={}
      settings: SourceProductName=ABB UPPAAL Library
  CB_51 : ABB_UPPAAL_Library/CB_1  MyInitialization=0  CB_ID=51  Sel_Type=3  m=3  i1=660  t1=170  i2_flag=off  i2=null  t2=null  i3_flag=off  i3=null  t3=null  i7=1320  t7FW=7  t7BW=7  tselFW=1  tselBW=1  Actors={ '44', '0', '0'; '46', '1', '0'; '50', '0', '1'; '52', '0', '0'; '53', '1', '1'; '57', '1', '1'; '62', '1', '1' }
      settings: SourceProductName=ABB UPPAAL Library
  CB_52 : ABB_UPPAAL_Library/CB_1  MyInitialization=0  CB_ID=52  Sel_Type=3  m=3  i1=900  t1=180  i2_flag=off  i2=null  t2=null  i3_flag=off  i3=null  t3=null  i7=1800  t7FW=8  t7BW=8  tselFW=1  tselBW=1  Actors={ '44', '0', '1'; '46', '1', '1'; '51', '1', '1' }
      settings: SourceProductName=ABB UPPAAL Library
  CB_53 : ABB_UPPAAL_Library/CB_1  MyInitialization=0  CB_ID=53  Sel_Type=1  m=3  i1=90  t1=160  i2_flag=on  i2=180  t2=6  i3_flag=off  i3=null  t3=null  i7=null  t7FW=null  t7BW=null  tselFW=null  tselBW=null  Actors={}
      settings: SourceProductName=ABB UPPAAL Library
  CB_54 : ABB_UPPAAL_Library/CB_1  MyInitialization=0  CB_ID=54  Sel_Type=1  m=3  i1=30  t1=100  i2_flag=on  i2=60  t2=2  i3_flag=off  i3=null  t3=null  i7=null  t7FW=null  t7BW=null  tselFW=null  tselBW=null  Actors={}
      settings: SourceProductName=ABB UPPAAL Library
  CB_55 : ABB_UPPAAL_Library/CB_1  MyInitialization=0  CB_ID=55  Sel_Type=1  m=3  i1=30  t1=100  i2_flag=on  i2=60  t2=2  i3_flag=off  i3=null  t3=null  i7=null  t7FW=null  t7BW=null  tselFW=null  tselBW=null  Actors={}
      settings: SourceProductName=ABB UPPAAL Library
  CB_56 : ABB_UPPAAL_Library/CB_1  MyInitialization=0  CB_ID=56  Sel_Type=1  m=3  i1=30  t1=100  i2_flag=on  i2=60  t2=2  i3_flag=off  i3=null  t3=null  i7=null  t7FW=null  t7BW=null  tselFW=null  tselBW=null  Actors={}
      settings: SourceProductName=ABB UPPAAL Library
  CB_57 : ABB_UPPAAL_Library/CB_1  MyInitialization=0  CB_ID=57  Sel_Type=1  m=3  i1=90  t1=160  i2_flag=on  i2=180  t2=6  i3_flag=off  i3=null  t3=null  i7=null  t7FW=null  t7BW=null  tselFW=null  tselBW=null  Actors={}
      settings: SourceProductName=ABB UPPAAL Library
  CB_58 : ABB_UPPAAL_Library/CB_1  MyInitialization=0  CB_ID=58  Sel_Type=1  m=3  i1=30  t1=100  i2_flag=on  i2=60  t2=2  i3_flag=off  i3=null  t3=null  i7=null  t7FW=null  t7BW=null  tselFW=null  tselBW=null  Actors={}
      settings: SourceProductName=ABB UPPAAL Library
  CB_59 : ABB_UPPAAL_Library/CB_1  MyInitialization=0  CB_ID=59  Sel_Type=1  m=3  i1=60  t1=120  i2_flag=on  i2=120  t2=4  i3_flag=off  i3=null  t3=null  i7=null  t7FW=null  t7BW=null  tselFW=null  tselBW=null  Actors={}
      settings: SourceProductName=ABB UPPAAL Library
  CB_6 : ABB_UPPAAL_Library/CB_1  MyInitialization=0  CB_ID=6  Sel_Type=1  m=3  i1=30  t1=100  i2_flag=on  i2=60  t2=2  i3_flag=off  i3=null  t3=null  i7=null  t7FW=null  t7BW=null  tselFW=null  tselBW=null  Actors={}
      settings: SourceProductName=ABB UPPAAL Library
  CB_60 : ABB_UPPAAL_Library/CB_1  MyInitialization=0  CB_ID=60  Sel_Type=1  m=3  i1=30  t1=100  i2_flag=on  i2=60  t2=2  i3_flag=off  i3=null  t3=null  i7=null  t7FW=null  t7BW=null  tselFW=null  tselBW=null  Actors={}
      settings: SourceProductName=ABB UPPAAL Library
  CB_61 : ABB_UPPAAL_Library/CB_1  MyInitialization=0  CB_ID=61  Sel_Type=1  m=3  i1=30  t1=100  i2_flag=on  i2=60  t2=2  i3_flag=off  i3=null  t3=null  i7=null  t7FW=null  t7BW=null  tselFW=null  tselBW=null  Actors={}
      settings: SourceProductName=ABB UPPAAL Library
  CB_62 : ABB_UPPAAL_Library/CB_1  MyInitialization=0  CB_ID=62  Sel_Type=1  m=3  i1=60  t1=120  i2_flag=on  i2=120  t2=4  i3_flag=off  i3=null  t3=null  i7=null  t7FW=null  t7BW=null  tselFW=null  tselBW=null  Actors={}
      settings: SourceProductName=ABB UPPAAL Library
  CB_63 : ABB_UPPAAL_Library/CB_1  MyInitialization=0  CB_ID=63  Sel_Type=1  m=3  i1=30  t1=100  i2_flag=on  i2=60  t2=2  i3_flag=off  i3=null  t3=null  i7=null  t7FW=null  t7BW=null  tselFW=null  tselBW=null  Actors={}
      settings: SourceProductName=ABB UPPAAL Library
  CB_64 : ABB_UPPAAL_Library/CB_1  MyInitialization=0  CB_ID=64  Sel_Type=1  m=3  i1=30  t1=100  i2_flag=on  i2=60  t2=2  i3_flag=off  i3=null  t3=null  i7=null  t7FW=null  t7BW=null  tselFW=null  tselBW=null  Actors={}
      settings: SourceProductName=ABB UPPAAL Library
  CB_7 : ABB_UPPAAL_Library/CB_1  MyInitialization=0  CB_ID=7  Sel_Type=1  m=3  i1=30  t1=100  i2_flag=on  i2=60  t2=2  i3_flag=off  i3=null  t3=null  i7=null  t7FW=null  t7BW=null  tselFW=null  tselBW=null  Actors={}
      settings: SourceProductName=ABB UPPAAL Library
  CB_8 : ABB_UPPAAL_Library/CB_1  MyInitialization=0  CB_ID=8  Sel_Type=3  m=3  i1=900  t1=180  i2_flag=off  i2=null  t2=null  i3_flag=off  i3=null  t3=null  i7=1800  t7FW=8  t7BW=8  tselFW=1  tselBW=1  Actors={ '9', '0', '1'; '10', '1', '1'; '15', '1', '1' }
      settings: SourceProductName=ABB UPPAAL Library
  CB_9 : ABB_UPPAAL_Library/CB_1  MyInitialization=0  CB_ID=9  Sel_Type=3  m=3  i1=810  t1=170  i2_flag=off  i2=null  t2=null  i3_flag=off  i3=null  t3=null  i7=1620  t7FW=7  t7BW=7  tselFW=1  tselBW=1  Actors={ '2', '0', '0'; '3', '0', '0'; '4', '1', '0'; '8', '0', '1'; '10', '1', '1'; '15', '1', '1' }
      settings: SourceProductName=ABB UPPAAL Library
  Line_1 : ABB_UPPAAL_Library/Line_1  MyInitialization=0  Line_ID=1  Iioc=75  Ith=900  Fault_flag=1
      settings: SourceProductName=ABB UPPAAL Library
  Line_10 : ABB_UPPAAL_Library/Line_1  MyInitialization=0  Line_ID=10  Iioc=75  Ith=90  Fault_flag=1
      settings: SourceProductName=ABB UPPAAL Library
  Line_11 : ABB_UPPAAL_Library/Line_1  MyInitialization=0  Line_ID=11  Iioc=25  Ith=30  Fault_flag=1
      settings: SourceProductName=ABB UPPAAL Library
  Line_12 : ABB_UPPAAL_Library/Line_1  MyInitialization=0  Line_ID=12  Iioc=50  Ith=60  Fault_flag=1
      settings: SourceProductName=ABB UPPAAL Library
  Line_13 : ABB_UPPAAL_Library/Line_1  MyInitialization=0  Line_ID=13  Iioc=25  Ith=30  Fault_flag=1
      settings: SourceProductName=ABB UPPAAL Library
  Line_14 : ABB_UPPAAL_Library/Line_1  MyInitialization=0  Line_ID=14  Iioc=25  Ith=30  Fault_flag=1
      settings: SourceProductName=ABB UPPAAL Library
  Line_15 : ABB_UPPAAL_Library/Line_1  MyInitialization=0  Line_ID=15  Iioc=75  Ith=720  Fault_flag=1
      settings: SourceProductName=ABB UPPAAL Library
  Line_16 : ABB_UPPAAL_Library/Line_1  MyInitialization=0  Line_ID=16  Iioc=75  Ith=900  Fault_flag=1
      settings: SourceProductName=ABB UPPAAL Library
  Line_17 : ABB_UPPAAL_Library/Line_1  MyInitialization=0  Line_ID=17  Iioc=75  Ith=90  Fault_flag=1
      settings: SourceProductName=ABB UPPAAL Library
  Line_18 : ABB_UPPAAL_Library/Line_1  MyInitialization=0  Line_ID=18  Iioc=25  Ith=30  Fault_flag=1
      settings: SourceProductName=ABB UPPAAL Library
  Line_19 : ABB_UPPAAL_Library/Line_1  MyInitialization=0  Line_ID=19  Iioc=25  Ith=30  Fault_flag=1
      settings: SourceProductName=ABB UPPAAL Library
  Line_2 : ABB_UPPAAL_Library/Line_1  MyInitialization=0  Line_ID=2  Iioc=75  Ith=900  Fault_flag=1
      settings: SourceProductName=ABB UPPAAL Library
  Line_20 : ABB_UPPAAL_Library/Line_1  MyInitialization=0  Line_ID=20  Iioc=25  Ith=30  Fault_flag=1
      settings: SourceProductName=ABB UPPAAL Library
  Line_21 : ABB_UPPAAL_Library/Line_1  MyInitialization=0  Line_ID=21  Iioc=75  Ith=900  Fault_flag=1
      settings: SourceProductName=ABB UPPAAL Library
  Line_22 : ABB_UPPAAL_Library/Line_1  MyInitialization=0  Line_ID=22  Iioc=75  Ith=630  Fault_flag=1
      settings: SourceProductName=ABB UPPAAL Library
  Line_23 : ABB_UPPAAL_Library/Line_1  MyInitialization=0  Line_ID=23  Iioc=75  Ith=90  Fault_flag=1
      settings: SourceProductName=ABB UPPAAL Library
  Line_24 : ABB_UPPAAL_Library/Line_1  MyInitialization=0  Line_ID=24  Iioc=25  Ith=30  Fault_flag=1
      settings: SourceProductName=ABB UPPAAL Library
  Line_25 : ABB_UPPAAL_Library/Line_1  MyInitialization=0  Line_ID=25  Iioc=50  Ith=60  Fault_flag=1
      settings: SourceProductName=ABB UPPAAL Library
  Line_26 : ABB_UPPAAL_Library/Line_1  MyInitialization=0  Line_ID=26  Iioc=25  Ith=30  Fault_flag=1
      settings: SourceProductName=ABB UPPAAL Library
  Line_27 : ABB_UPPAAL_Library/Line_1  MyInitialization=0  Line_ID=27  Iioc=25  Ith=30  Fault_flag=1
      settings: SourceProductName=ABB UPPAAL Library
  Line_28 : ABB_UPPAAL_Library/Line_1  MyInitialization=0  Line_ID=28  Iioc=125  Ith=310  Fault_flag=1
      settings: SourceProductName=ABB UPPAAL Library
  Line_29 : ABB_UPPAAL_Library/Line_1  MyInitialization=0  Line_ID=29  Iioc=75  Ith=900  Fault_flag=1
      settings: SourceProductName=ABB UPPAAL Library
  Line_3 : ABB_UPPAAL_Library/Line_1  MyInitialization=0  Line_ID=3  Iioc=75  Ith=900  Fault_flag=1
      settings: SourceProductName=ABB UPPAAL Library
  Line_30 : ABB_UPPAAL_Library/Line_1  MyInitialization=0  Line_ID=30  Iioc=125  Ith=600  Fault_flag=1
      settings: SourceProductName=ABB UPPAAL Library
  Line_31 : ABB_UPPAAL_Library/Line_1  MyInitialization=0  Line_ID=31  Iioc=25  Ith=30  Fault_flag=1
      settings: SourceProductName=ABB UPPAAL Library
  Line_32 : ABB_UPPAAL_Library/Line_1  MyInitialization=0  Line_ID=32  Iioc=75  Ith=90  Fault_flag=1
      settings: SourceProductName=ABB UPPAAL Library
  Line_33 : ABB_UPPAAL_Library/Line_1  MyInitialization=0  Line_ID=33  Iioc=25  Ith=30  Fault_flag=1
      settings: SourceProductName=ABB UPPAAL Library
  Line_34 : ABB_UPPAAL_Library/Line_1  MyInitialization=0  Line_ID=34  Iioc=50  Ith=60  Fault_flag=1
      settings: SourceProductName=ABB UPPAAL Library
  Line_35 : ABB_UPPAAL_Library/Line_1  MyInitialization=0  Line_ID=35  Iioc=25  Ith=30  Fault_flag=1
      settings: SourceProductName=ABB UPPAAL Library
  Line_36 : ABB_UPPAAL_Library/Line_1  MyInitialization=0  Line_ID=36  Iioc=25  Ith=30  Fault_flag=1
      settings: SourceProductName=ABB UPPAAL Library
  Line_37 : ABB_UPPAAL_Library/Line_1  MyInitialization=0  Line_ID=37  Iioc=125  Ith=480  Fault_flag=1
      settings: SourceProductName=ABB UPPAAL Library
  Line_38 : ABB_UPPAAL_Library/Line_1  MyInitialization=0  Line_ID=38  Iioc=75  Ith=900  Fault_flag=1
      settings: SourceProductName=ABB UPPAAL Library
  Line_39 : ABB_UPPAAL_Library/Line_1  MyInitialization=0  Line_ID=39  Iioc=75  Ith=90  Fault_flag=1
      settings: SourceProductName=ABB UPPAAL Library
  Line_4 : ABB_UPPAAL_Library/Line_1  MyInitialization=0  Line_ID=4  Iioc=75  Ith=90  Fault_flag=1
      settings: SourceProductName=ABB UPPAAL Library
  Line_40 : ABB_UPPAAL_Library/Line_1  MyInitialization=0  Line_ID=40  Iioc=25  Ith=30  Fault_flag=1
      settings: SourceProductName=ABB UPPAAL Library
  Line_41 : ABB_UPPAAL_Library/Line_1  MyInitialization=0  Line_ID=41  Iioc=50  Ith=60  Fault_flag=1
      settings: SourceProductName=ABB UPPAAL Library
  Line_42 : ABB_UPPAAL_Library/Line_1  MyInitialization=0  Line_ID=42  Iioc=25  Ith=30  Fault_flag=1
      settings: SourceProductName=ABB UPPAAL Library
  Line_43 : ABB_UPPAAL_Library/Line_1  MyInitialization=0  Line_ID=43  Iioc=25  Ith=30  Fault_flag=1
      settings: SourceProductName=ABB UPPAAL Library
  Line_44 : ABB_UPPAAL_Library/Line_1  MyInitialization=0  Line_ID=44  Iioc=125  Ith=570  Fault_flag=1
      settings: SourceProductName=ABB UPPAAL Library
  Line_45 : ABB_UPPAAL_Library/Line_1  MyInitialization=0  Line_ID=45  Iioc=75  Ith=900  Fault_flag=1
      settings: SourceProductName=ABB UPPAAL Library
  Line_46 : ABB_UPPAAL_Library/Line_1  MyInitialization=0  Line_ID=46  Iioc=75  Ith=90  Fault_flag=1
      settings: SourceProductName=ABB UPPAAL Library
  Line_47 : ABB_UPPAAL_Library/Line_1  MyInitialization=0  Line_ID=47  Iioc=25  Ith=30  Fault_flag=1
      settings: SourceProductName=ABB UPPAAL Library
  Line_48 : ABB_UPPAAL_Library/Line_1  MyInitialization=0  Line_ID=48  Iioc=25  Ith=30  Fault_flag=1
      settings: SourceProductName=ABB UPPAAL Library
  Line_49 : ABB_UPPAAL_Library/Line_1  MyInitialization=0  Line_ID=49  Iioc=25  Ith=30  Fault_flag=1
      settings: SourceProductName=ABB UPPAAL Library
  Line_5 : ABB_UPPAAL_Library/Line_1  MyInitialization=0  Line_ID=5  Iioc=25  Ith=30  Fault_flag=1
      settings: SourceProductName=ABB UPPAAL Library
  Line_50 : ABB_UPPAAL_Library/Line_1  MyInitialization=0  Line_ID=50  Iioc=75  Ith=900  Fault_flag=1
      settings: SourceProductName=ABB UPPAAL Library
  Line_51 : ABB_UPPAAL_Library/Line_1  MyInitialization=0  Line_ID=51  Iioc=125  Ith=660  Fault_flag=1
      settings: SourceProductName=ABB UPPAAL Library
  Line_52 : ABB_UPPAAL_Library/Line_1  MyInitialization=0  Line_ID=52  Iioc=75  Ith=900  Fault_flag=1
      settings: SourceProductName=ABB UPPAAL Library
  Line_53 : ABB_UPPAAL_Library/Line_1  MyInitialization=0  Line_ID=53  Iioc=75  Ith=90  Fault_flag=1
      settings: SourceProductName=ABB UPPAAL Library
  Line_54 : ABB_UPPAAL_Library/Line_1  MyInitialization=0  Line_ID=54  Iioc=25  Ith=30  Fault_flag=1
      settings: SourceProductName=ABB UPPAAL Library
  Line_55 : ABB_UPPAAL_Library/Line_1  MyInitialization=0  Line_ID=55  Iioc=25  Ith=30  Fault_flag=1
      settings: SourceProductName=ABB UPPAAL Library
  Line_56 : ABB_UPPAAL_Library/Line_1  MyInitialization=0  Line_ID=56  Iioc=25  Ith=30  Fault_flag=1
      settings: SourceProductName=ABB UPPAAL Library
  Line_57 : ABB_UPPAAL_Library/Line_1  MyInitialization=0  Line_ID=57  Iioc=75  Ith=90  Fault_flag=1
      settings: SourceProductName=ABB UPPAAL Library
  Line_58 : ABB_UPPAAL_Library/Line_1  MyInitialization=0  Line_ID=58  Iioc=25  Ith=30  Fault_flag=1
      settings: SourceProductName=ABB UPPAAL Library
  Line_59 : ABB_UPPAAL_Library/Line_1  MyInitialization=0  Line_ID=59  Iioc=50  Ith=60  Fault_flag=1
      settings: SourceProductName=ABB UPPAAL Library
  Line_6 : ABB_UPPAAL_Library/Line_1  MyInitialization=0  Line_ID=6  Iioc=25  Ith=30  Fault_flag=1
      settings: SourceProductName=ABB UPPAAL Library
  Line_60 : ABB_UPPAAL_Library/Line_1  MyInitialization=0  Line_ID=60  Iioc=25  Ith=30  Fault_flag=1
      settings: SourceProductName=ABB UPPAAL Library
  Line_61 : ABB_UPPAAL_Library/Line_1  MyInitialization=0  Line_ID=61  Iioc=25  Ith=30  Fault_flag=1
      settings: SourceProductName=ABB UPPAAL Library
  Line_62 : ABB_UPPAAL_Library/Line_1  MyInitialization=0  Line_ID=62  Iioc=50  Ith=60  Fault_flag=1
      settings: SourceProductName=ABB UPPAAL Library
  Line_63 : ABB_UPPAAL_Library/Line_1  MyInitialization=0  Line_ID=63  Iioc=25  Ith=30  Fault_flag=1
      settings: SourceProductName=ABB UPPAAL Library
  Line_64 : ABB_UPPAAL_Library/Line_1  MyInitialization=0  Line_ID=64  Iioc=25  Ith=30  Fault_flag=1
      settings: SourceProductName=ABB UPPAAL Library
  Line_7 : ABB_UPPAAL_Library/Line_1  MyInitialization=0  Line_ID=7  Iioc=25  Ith=30  Fault_flag=1
      settings: SourceProductName=ABB UPPAAL Library
  Line_8 : ABB_UPPAAL_Library/Line_1  MyInitialization=0  Line_ID=8  Iioc=75  Ith=900  Fault_flag=1
      settings: SourceProductName=ABB UPPAAL Library
  Line_9 : ABB_UPPAAL_Library/Line_1  MyInitialization=0  Line_ID=9  Iioc=75  Ith=810  Fault_flag=1
      settings: SourceProductName=ABB UPPAAL Library
  Load_1 : ABB_UPPAAL_Library/Load_1  MyInitialization=0  Load_ID=1
      settings: SourceProductName=ABB UPPAAL Library
  Load_10 : ABB_UPPAAL_Library/Load_1  MyInitialization=0  Load_ID=10
      settings: SourceProductName=ABB UPPAAL Library
  Load_11 : ABB_UPPAAL_Library/Load_1  MyInitialization=0  Load_ID=11
      settings: SourceProductName=ABB UPPAAL Library
  Load_12 : ABB_UPPAAL_Library/Load_1  MyInitialization=0  Load_ID=12
      settings: SourceProductName=ABB UPPAAL Library
  Load_13 : ABB_UPPAAL_Library/Load_1  MyInitialization=0  Load_ID=13
      settings: SourceProductName=ABB UPPAAL Library
  Load_14 : ABB_UPPAAL_Library/Load_1  MyInitialization=0  Load_ID=14
      settings: SourceProductName=ABB UPPAAL Library
  Load_15 : ABB_UPPAAL_Library/Load_1  MyInitialization=0  Load_ID=15
      settings: SourceProductName=ABB UPPAAL Library
  Load_16 : ABB_UPPAAL_Library/Load_1  MyInitialization=0  Load_ID=16
      settings: SourceProductName=ABB UPPAAL Library
  Load_17 : ABB_UPPAAL_Library/Load_1  MyInitialization=0  Load_ID=17
      settings: SourceProductName=ABB UPPAAL Library
  Load_18 : ABB_UPPAAL_Library/Load_1  MyInitialization=0  Load_ID=18
      settings: SourceProductName=ABB UPPAAL Library
  Load_19 : ABB_UPPAAL_Library/Load_1  MyInitialization=0  Load_ID=19
      settings: SourceProductName=ABB UPPAAL Library
  Load_2 : ABB_UPPAAL_Library/Load_1  MyInitialization=0  Load_ID=2
      settings: SourceProductName=ABB UPPAAL Library
  Load_20 : ABB_UPPAAL_Library/Load_1  MyInitialization=0  Load_ID=20
      settings: SourceProductName=ABB UPPAAL Library
  Load_21 : ABB_UPPAAL_Library/Load_1  MyInitialization=0  Load_ID=21
      settings: SourceProductName=ABB UPPAAL Library
  Load_22 : ABB_UPPAAL_Library/Load_1  MyInitialization=0  Load_ID=22
      settings: SourceProductName=ABB UPPAAL Library
  Load_23 : ABB_UPPAAL_Library/Load_1  MyInitialization=0  Load_ID=23
      settings: SourceProductName=ABB UPPAAL Library
  Load_24 : ABB_UPPAAL_Library/Load_1  MyInitialization=0  Load_ID=24
      settings: SourceProductName=ABB UPPAAL Library
  Load_25 : ABB_UPPAAL_Library/Load_1  MyInitialization=0  Load_ID=25
      settings: SourceProductName=ABB UPPAAL Library
  Load_26 : ABB_UPPAAL_Library/Load_1  MyInitialization=0  Load_ID=26
      settings: SourceProductName=ABB UPPAAL Library
  Load_27 : ABB_UPPAAL_Library/Load_1  MyInitialization=0  Load_ID=27
      settings: SourceProductName=ABB UPPAAL Library
  Load_28 : ABB_UPPAAL_Library/Load_1  MyInitialization=0  Load_ID=28
      settings: SourceProductName=ABB UPPAAL Library
  Load_29 : ABB_UPPAAL_Library/Load_1  MyInitialization=0  Load_ID=29
      settings: SourceProductName=ABB UPPAAL Library
  Load_3 : ABB_UPPAAL_Library/Load_1  MyInitialization=0  Load_ID=3
      settings: SourceProductName=ABB UPPAAL Library
  Load_30 : ABB_UPPAAL_Library/Load_1  MyInitialization=0  Load_ID=30
      settings: SourceProductName=ABB UPPAAL Library
  Load_4 : ABB_UPPAAL_Library/Load_1  MyInitialization=0  Load_ID=4
      settings: SourceProductName=ABB UPPAAL Library
  Load_5 : ABB_UPPAAL_Library/Load_1  MyInitialization=0  Load_ID=5
      settings: SourceProductName=ABB UPPAAL Library
  Load_6 : ABB_UPPAAL_Library/Load_1  MyInitialization=0  Load_ID=6
      settings: SourceProductName=ABB UPPAAL Library
  Load_7 : ABB_UPPAAL_Library/Load_1  MyInitialization=0  Load_ID=7
      settings: SourceProductName=ABB UPPAAL Library
  Load_8 : ABB_UPPAAL_Library/Load_1  MyInitialization=0  Load_ID=8
      settings: SourceProductName=ABB UPPAAL Library
  Load_9 : ABB_UPPAAL_Library/Load_1  MyInitialization=0  Load_ID=9
      settings: SourceProductName=ABB UPPAAL Library
  Source_1 : ABB_UPPAAL_Library/Source_1  MyInitialization=0  Source_ID=1  Lines_Isc={ '1', '1000'; '2', '1000'; '3', '1000'; '4', '1000'; '5', '1000'; '6', '1000'; '7', '1000'; '8', '1000'; '9', '1000'; '10', '1000'; '11', '1000'; '12', '1000'; '13', '1000'; '14', '1000'; '15', '1000'; '16', '1000'; '17', '1000'; '18', '1000'; '19', '1000'; '20', '1000'; '21', '1000'; '22', '1000'; '23', '1000'; '24', '1000'; '25', '1000'; '26', '1000'; '27', '1000'; '28', '1000'; '29', '1000'; '30', '1000'; '31', '1000'; '32', '1000'; '33', '1000'; '34', '1000'; '35', '1000'; '36', '1000'; '37', '1000'; '38', '1000'; '39', '1000'; '40', '1000'; '41', '1000'; '42', '1000'; '43', '1000'; '44', '1000'; '45', '1000'; '46', '1000'; '47', '1000'; '48', '1000'; '49', '1000'; '50', '1000'; '51', '1000'; '52', '1000'; '53', '1000'; '54', '1000'; '55', '1000'; '56', '1000'; '57', '1000'; '58', '1000'; '59', '1000'; '60', '1000'; '61', '1000'; '62', '1000'; '63', '1000'; '64', '1000' }  Buses_Isc={ '1', '1000'; '2', '1000'; '3', '1000'; '4', '1000'; '5', '1000'; '6', '1000'; '7', '1000'; '8', '1000'; '9', '1000'; '10', '1000'; '11', '1000'; '12', '1000'; '13', '1000'; '14', '1000'; '15', '1000'; '16', '1000'; '17', '1000'; '18', '1000'; '19', '1000'; '20', '1000'; '21', '1000'; '22', '1000'; '23', '1000'; '24', '1000'; '25', '1000'; '26', '1000'; '27', '1000'; '28', '1000'; '29', '1000'; '30', '1000'; '31', '1000'; '32', '1000'; '33', '1000'; '34', '1000'; '35', '1000'; '36', '1000'; '37', '1000'; '38', '1000'; '39', '1000'; '40', '1000'; '41', '1000'; '42', '1000'; '43', '1000'; '44', '1000'; '45', '1000'; '46', '1000'; '47', '1000'; '48', '1000'; '49', '1000'; '50', '1000'; '51', '1000'; '52', '1000'; '53', '1000'; '54', '1000'; '55', '1000'; '56', '1000'; '57', '1000'; '58', '1000'; '59', '1000'; '60', '1000'; '61', '1000'; '62', '1000'; '63', '1000'; '64', '1000'; '65', '1000' }
      settings: SourceProductName=ABB UPPAAL Library
  Source_16 : ABB_UPPAAL_Library/Source_1  MyInitialization=0  Source_ID=16  Lines_Isc={ '1', '1000'; '2', '1000'; '3', '1000'; '4', '1000'; '5', '1000'; '6', '1000'; '7', '1000'; '8', '1000'; '9', '1000'; '10', '1000'; '11', '1000'; '12', '1000'; '13', '1000'; '14', '1000'; '15', '1000'; '16', '1000'; '17', '1000'; '18', '1000'; '19', '1000'; '20', '1000'; '21', '1000'; '22', '1000'; '23', '1000'; '24', '1000'; '25', '1000'; '26', '1000'; '27', '1000'; '28', '1000'; '29', '1000'; '30', '1000'; '31', '1000'; '32', '1000'; '33', '1000'; '34', '1000'; '35', '1000'; '36', '1000'; '37', '1000'; '38', '1000'; '39', '1000'; '40', '1000'; '41', '1000'; '42', '1000'; '43', '1000'; '44', '1000'; '45', '1000'; '46', '1000'; '47', '1000'; '48', '1000'; '49', '1000'; '50', '1000'; '51', '1000'; '52', '1000'; '53', '1000'; '54', '1000'; '55', '1000'; '56', '1000'; '57', '1000'; '58', '1000'; '59', '1000'; '60', '1000'; '61', '1000'; '62', '1000'; '63', '1000'; '64', '1000' }  Buses_Isc={ '1', '1000'; '2', '1000'; '3', '1000'; '4', '1000'; '5', '1000'; '6', '1000'; '7', '1000'; '8', '1000'; '9', '1000'; '10', '1000'; '11', '1000'; '12', '1000'; '13', '1000'; '14', '1000'; '15', '1000'; '16', '1000'; '17', '1000'; '18', '1000'; '19', '1000'; '20', '1000'; '21', '1000'; '22', '1000'; '23', '1000'; '24', '1000'; '25', '1000'; '26', '1000'; '27', '1000'; '28', '1000'; '29', '1000'; '30', '1000'; '31', '1000'; '32', '1000'; '33', '1000'; '34', '1000'; '35', '1000'; '36', '1000'; '37', '1000'; '38', '1000'; '39', '1000'; '40', '1000'; '41', '1000'; '42', '1000'; '43', '1000'; '44', '1000'; '45', '1000'; '46', '1000'; '47', '1000'; '48', '1000'; '49', '1000'; '50', '1000'; '51', '1000'; '52', '1000'; '53', '1000'; '54', '1000'; '55', '1000'; '56', '1000'; '57', '1000'; '58', '1000'; '59', '1000'; '60', '1000'; '61', '1000'; '62', '1000'; '63', '1000'; '64', '1000'; '65', '1000' }
      settings: SourceProductName=ABB UPPAAL Library
  Source_2 : ABB_UPPAAL_Library/Source_1  MyInitialization=0  Source_ID=2  Lines_Isc={ '1', '1000'; '2', '1000'; '3', '1000'; '4', '1000'; '5', '1000'; '6', '1000'; '7', '1000'; '8', '1000'; '9', '1000'; '10', '1000'; '11', '1000'; '12', '1000'; '13', '1000'; '14', '1000'; '15', '1000'; '16', '1000'; '17', '1000'; '18', '1000'; '19', '1000'; '20', '1000'; '21', '1000'; '22', '1000'; '23', '1000'; '24', '1000'; '25', '1000'; '26', '1000'; '27', '1000'; '28', '1000'; '29', '1000'; '30', '1000'; '31', '1000'; '32', '1000'; '33', '1000'; '34', '1000'; '35', '1000'; '36', '1000'; '37', '1000'; '38', '1000'; '39', '1000'; '40', '1000'; '41', '1000'; '42', '1000'; '43', '1000'; '44', '1000'; '45', '1000'; '46', '1000'; '47', '1000'; '48', '1000'; '49', '1000'; '50', '1000'; '51', '1000'; '52', '1000'; '53', '1000'; '54', '1000'; '55', '1000'; '56', '1000'; '57', '1000'; '58', '1000'; '59', '1000'; '60', '1000'; '61', '1000'; '62', '1000'; '63', '1000'; '64', '1000' }  Buses_Isc={ '1', '1000'; '2', '1000'; '3', '1000'; '4', '1000'; '5', '1000'; '6', '1000'; '7', '1000'; '8', '1000'; '9', '1000'; '10', '1000'; '11', '1000'; '12', '1000'; '13', '1000'; '14', '1000'; '15', '1000'; '16', '1000'; '17', '1000'; '18', '1000'; '19', '1000'; '20', '1000'; '21', '1000'; '22', '1000'; '23', '1000'; '24', '1000'; '25', '1000'; '26', '1000'; '27', '1000'; '28', '1000'; '29', '1000'; '30', '1000'; '31', '1000'; '32', '1000'; '33', '1000'; '34', '1000'; '35', '1000'; '36', '1000'; '37', '1000'; '38', '1000'; '39', '1000'; '40', '1000'; '41', '1000'; '42', '1000'; '43', '1000'; '44', '1000'; '45', '1000'; '46', '1000'; '47', '1000'; '48', '1000'; '49', '1000'; '50', '1000'; '51', '1000'; '52', '1000'; '53', '1000'; '54', '1000'; '55', '1000'; '56', '1000'; '57', '1000'; '58', '1000'; '59', '1000'; '60', '1000'; '61', '1000'; '62', '1000'; '63', '1000'; '64', '1000'; '65', '1000' }
      settings: SourceProductName=ABB UPPAAL Library
  Source_22 : ABB_UPPAAL_Library/Source_1  MyInitialization=0  Source_ID=22  Lines_Isc={ '1', '1000'; '2', '1000'; '3', '1000'; '4', '1000'; '5', '1000'; '6', '1000'; '7', '1000'; '8', '1000'; '9', '1000'; '10', '1000'; '11', '1000'; '12', '1000'; '13', '1000'; '14', '1000'; '15', '1000'; '16', '1000'; '17', '1000'; '18', '1000'; '19', '1000'; '20', '1000'; '21', '1000'; '22', '1000'; '23', '1000'; '24', '1000'; '25', '1000'; '26', '1000'; '27', '1000'; '28', '1000'; '29', '1000'; '30', '1000'; '31', '1000'; '32', '1000'; '33', '1000'; '34', '1000'; '35', '1000'; '36', '1000'; '37', '1000'; '38', '1000'; '39', '1000'; '40', '1000'; '41', '1000'; '42', '1000'; '43', '1000'; '44', '1000'; '45', '1000'; '46', '1000'; '47', '1000'; '48', '1000'; '49', '1000'; '50', '1000'; '51', '1000'; '52', '1000'; '53', '1000'; '54', '1000'; '55', '1000'; '56', '1000'; '57', '1000'; '58', '1000'; '59', '1000'; '60', '1000'; '61', '1000'; '62', '1000'; '63', '1000'; '64', '1000' }  Buses_Isc={ '1', '1000'; '2', '1000'; '3', '1000'; '4', '1000'; '5', '1000'; '6', '1000'; '7', '1000'; '8', '1000'; '9', '1000'; '10', '1000'; '11', '1000'; '12', '1000'; '13', '1000'; '14', '1000'; '15', '1000'; '16', '1000'; '17', '1000'; '18', '1000'; '19', '1000'; '20', '1000'; '21', '1000'; '22', '1000'; '23', '1000'; '24', '1000'; '25', '1000'; '26', '1000'; '27', '1000'; '28', '1000'; '29', '1000'; '30', '1000'; '31', '1000'; '32', '1000'; '33', '1000'; '34', '1000'; '35', '1000'; '36', '1000'; '37', '1000'; '38', '1000'; '39', '1000'; '40', '1000'; '41', '1000'; '42', '1000'; '43', '1000'; '44', '1000'; '45', '1000'; '46', '1000'; '47', '1000'; '48', '1000'; '49', '1000'; '50', '1000'; '51', '1000'; '52', '1000'; '53', '1000'; '54', '1000'; '55', '1000'; '56', '1000'; '57', '1000'; '58', '1000'; '59', '1000'; '60', '1000'; '61', '1000'; '62', '1000'; '63', '1000'; '64', '1000'; '65', '1000' }
      settings: SourceProductName=ABB UPPAAL Library
  Source_31 : ABB_UPPAAL_Library/Source_1  MyInitialization=0  Source_ID=31  Lines_Isc={ '1', '1000'; '2', '1000'; '3', '1000'; '4', '1000'; '5', '1000'; '6', '1000'; '7', '1000'; '8', '1000'; '9', '1000'; '10', '1000'; '11', '1000'; '12', '1000'; '13', '1000'; '14', '1000'; '15', '1000'; '16', '1000'; '17', '1000'; '18', '1000'; '19', '1000'; '20', '1000'; '21', '1000'; '22', '1000'; '23', '1000'; '24', '1000'; '25', '1000'; '26', '1000'; '27', '1000'; '28', '1000'; '29', '1000'; '30', '1000'; '31', '1000'; '32', '1000'; '33', '1000'; '34', '1000'; '35', '1000'; '36', '1000'; '37', '1000'; '38', '1000'; '39', '1000'; '40', '1000'; '41', '1000'; '42', '1000'; '43', '1000'; '44', '1000'; '45', '1000'; '46', '1000'; '47', '1000'; '48', '1000'; '49', '1000'; '50', '1000'; '51', '1000'; '52', '1000'; '53', '1000'; '54', '1000'; '55', '1000'; '56', '1000'; '57', '1000'; '58', '1000'; '59', '1000'; '60', '1000'; '61', '1000'; '62', '1000'; '63', '1000'; '64', '1000' }  Buses_Isc={ '1', '1000'; '2', '1000'; '3', '1000'; '4', '1000'; '5', '1000'; '6', '1000'; '7', '1000'; '8', '1000'; '9', '1000'; '10', '1000'; '11', '1000'; '12', '1000'; '13', '1000'; '14', '1000'; '15', '1000'; '16', '1000'; '17', '1000'; '18', '1000'; '19', '1000'; '20', '1000'; '21', '1000'; '22', '1000'; '23', '1000'; '24', '1000'; '25', '1000'; '26', '1000'; '27', '1000'; '28', '1000'; '29', '1000'; '30', '1000'; '31', '1000'; '32', '1000'; '33', '1000'; '34', '1000'; '35', '1000'; '36', '1000'; '37', '1000'; '38', '1000'; '39', '1000'; '40', '1000'; '41', '1000'; '42', '1000'; '43', '1000'; '44', '1000'; '45', '1000'; '46', '1000'; '47', '1000'; '48', '1000'; '49', '1000'; '50', '1000'; '51', '1000'; '52', '1000'; '53', '1000'; '54', '1000'; '55', '1000'; '56', '1000'; '57', '1000'; '58', '1000'; '59', '1000'; '60', '1000'; '61', '1000'; '62', '1000'; '63', '1000'; '64', '1000'; '65', '1000' }
      settings: SourceProductName=ABB UPPAAL Library
  Source_38 : ABB_UPPAAL_Library/Source_1  MyInitialization=0  Source_ID=38  Lines_Isc={ '1', '1000'; '2', '1000'; '3', '1000'; '4', '1000'; '5', '1000'; '6', '1000'; '7', '1000'; '8', '1000'; '9', '1000'; '10', '1000'; '11', '1000'; '12', '1000'; '13', '1000'; '14', '1000'; '15', '1000'; '16', '1000'; '17', '1000'; '18', '1000'; '19', '1000'; '20', '1000'; '21', '1000'; '22', '1000'; '23', '1000'; '24', '1000'; '25', '1000'; '26', '1000'; '27', '1000'; '28', '1000'; '29', '1000'; '30', '1000'; '31', '1000'; '32', '1000'; '33', '1000'; '34', '1000'; '35', '1000'; '36', '1000'; '37', '1000'; '38', '1000'; '39', '1000'; '40', '1000'; '41', '1000'; '42', '1000'; '43', '1000'; '44', '1000'; '45', '1000'; '46', '1000'; '47', '1000'; '48', '1000'; '49', '1000'; '50', '1000'; '51', '1000'; '52', '1000'; '53', '1000'; '54', '1000'; '55', '1000'; '56', '1000'; '57', '1000'; '58', '1000'; '59', '1000'; '60', '1000'; '61', '1000'; '62', '1000'; '63', '1000'; '64', '1000' }  Buses_Isc={ '1', '1000'; '2', '1000'; '3', '1000'; '4', '1000'; '5', '1000'; '6', '1000'; '7', '1000'; '8', '1000'; '9', '1000'; '10', '1000'; '11', '1000'; '12', '1000'; '13', '1000'; '14', '1000'; '15', '1000'; '16', '1000'; '17', '1000'; '18', '1000'; '19', '1000'; '20', '1000'; '21', '1000'; '22', '1000'; '23', '1000'; '24', '1000'; '25', '1000'; '26', '1000'; '27', '1000'; '28', '1000'; '29', '1000'; '30', '1000'; '31', '1000'; '32', '1000'; '33', '1000'; '34', '1000'; '35', '1000'; '36', '1000'; '37', '1000'; '38', '1000'; '39', '1000'; '40', '1000'; '41', '1000'; '42', '1000'; '43', '1000'; '44', '1000'; '45', '1000'; '46', '1000'; '47', '1000'; '48', '1000'; '49', '1000'; '50', '1000'; '51', '1000'; '52', '1000'; '53', '1000'; '54', '1000'; '55', '1000'; '56', '1000'; '57', '1000'; '58', '1000'; '59', '1000'; '60', '1000'; '61', '1000'; '62', '1000'; '63', '1000'; '64', '1000'; '65', '1000' }
      settings: SourceProductName=ABB UPPAAL Library
  Source_45 : ABB_UPPAAL_Library/Source_1  MyInitialization=0  Source_ID=45  Lines_Isc={ '1', '1000'; '2', '1000'; '3', '1000'; '4', '1000'; '5', '1000'; '6', '1000'; '7', '1000'; '8', '1000'; '9', '1000'; '10', '1000'; '11', '1000'; '12', '1000'; '13', '1000'; '14', '1000'; '15', '1000'; '16', '1000'; '17', '1000'; '18', '1000'; '19', '1000'; '20', '1000'; '21', '1000'; '22', '1000'; '23', '1000'; '24', '1000'; '25', '1000'; '26', '1000'; '27', '1000'; '28', '1000'; '29', '1000'; '30', '1000'; '31', '1000'; '32', '1000'; '33', '1000'; '34', '1000'; '35', '1000'; '36', '1000'; '37', '1000'; '38', '1000'; '39', '1000'; '40', '1000'; '41', '1000'; '42', '1000'; '43', '1000'; '44', '1000'; '45', '1000'; '46', '1000'; '47', '1000'; '48', '1000'; '49', '1000'; '50', '1000'; '51', '1000'; '52', '1000'; '53', '1000'; '54', '1000'; '55', '1000'; '56', '1000'; '57', '1000'; '58', '1000'; '59', '1000'; '60', '1000'; '61', '1000'; '62', '1000'; '63', '1000'; '64', '1000' }  Buses_Isc={ '1', '1000'; '2', '1000'; '3', '1000'; '4', '1000'; '5', '1000'; '6', '1000'; '7', '1000'; '8', '1000'; '9', '1000'; '10', '1000'; '11', '1000'; '12', '1000'; '13', '1000'; '14', '1000'; '15', '1000'; '16', '1000'; '17', '1000'; '18', '1000'; '19', '1000'; '20', '1000'; '21', '1000'; '22', '1000'; '23', '1000'; '24', '1000'; '25', '1000'; '26', '1000'; '27', '1000'; '28', '1000'; '29', '1000'; '30', '1000'; '31', '1000'; '32', '1000'; '33', '1000'; '34', '1000'; '35', '1000'; '36', '1000'; '37', '1000'; '38', '1000'; '39', '1000'; '40', '1000'; '41', '1000'; '42', '1000'; '43', '1000'; '44', '1000'; '45', '1000'; '46', '1000'; '47', '1000'; '48', '1000'; '49', '1000'; '50', '1000'; '51', '1000'; '52', '1000'; '53', '1000'; '54', '1000'; '55', '1000'; '56', '1000'; '57', '1000'; '58', '1000'; '59', '1000'; '60', '1000'; '61', '1000'; '62', '1000'; '63', '1000'; '64', '1000'; '65', '1000' }
      settings: SourceProductName=ABB UPPAAL Library
  Source_52 : ABB_UPPAAL_Library/Source_1  MyInitialization=0  Source_ID=52  Lines_Isc={ '1', '1000'; '2', '1000'; '3', '1000'; '4', '1000'; '5', '1000'; '6', '1000'; '7', '1000'; '8', '1000'; '9', '1000'; '10', '1000'; '11', '1000'; '12', '1000'; '13', '1000'; '14', '1000'; '15', '1000'; '16', '1000'; '17', '1000'; '18', '1000'; '19', '1000'; '20', '1000'; '21', '1000'; '22', '1000'; '23', '1000'; '24', '1000'; '25', '1000'; '26', '1000'; '27', '1000'; '28', '1000'; '29', '1000'; '30', '1000'; '31', '1000'; '32', '1000'; '33', '1000'; '34', '1000'; '35', '1000'; '36', '1000'; '37', '1000'; '38', '1000'; '39', '1000'; '40', '1000'; '41', '1000'; '42', '1000'; '43', '1000'; '44', '1000'; '45', '1000'; '46', '1000'; '47', '1000'; '48', '1000'; '49', '1000'; '50', '1000'; '51', '1000'; '52', '1000'; '53', '1000'; '54', '1000'; '55', '1000'; '56', '1000'; '57', '1000'; '58', '1000'; '59', '1000'; '60', '1000'; '61', '1000'; '62', '1000'; '63', '1000'; '64', '1000' }  Buses_Isc={ '1', '1000'; '2', '1000'; '3', '1000'; '4', '1000'; '5', '1000'; '6', '1000'; '7', '1000'; '8', '1000'; '9', '1000'; '10', '1000'; '11', '1000'; '12', '1000'; '13', '1000'; '14', '1000'; '15', '1000'; '16', '1000'; '17', '1000'; '18', '1000'; '19', '1000'; '20', '1000'; '21', '1000'; '22', '1000'; '23', '1000'; '24', '1000'; '25', '1000'; '26', '1000'; '27', '1000'; '28', '1000'; '29', '1000'; '30', '1000'; '31', '1000'; '32', '1000'; '33', '1000'; '34', '1000'; '35', '1000'; '36', '1000'; '37', '1000'; '38', '1000'; '39', '1000'; '40', '1000'; '41', '1000'; '42', '1000'; '43', '1000'; '44', '1000'; '45', '1000'; '46', '1000'; '47', '1000'; '48', '1000'; '49', '1000'; '50', '1000'; '51', '1000'; '52', '1000'; '53', '1000'; '54', '1000'; '55', '1000'; '56', '1000'; '57', '1000'; '58', '1000'; '59', '1000'; '60', '1000'; '61', '1000'; '62', '1000'; '63', '1000'; '64', '1000'; '65', '1000' }
      settings: SourceProductName=ABB UPPAAL Library
  Source_53 : ABB_UPPAAL_Library/Source_1  MyInitialization=0  Source_ID=53  Lines_Isc={ '1', '1000'; '2', '1000'; '3', '1000'; '4', '1000'; '5', '1000'; '6', '1000'; '7', '1000'; '8', '1000'; '9', '1000'; '10', '1000'; '11', '1000'; '12', '1000'; '13', '1000'; '14', '1000'; '15', '1000'; '16', '1000'; '17', '1000'; '18', '1000'; '19', '1000'; '20', '1000'; '21', '1000'; '22', '1000'; '23', '1000'; '24', '1000'; '25', '1000'; '26', '1000'; '27', '1000'; '28', '1000'; '29', '1000'; '30', '1000'; '31', '1000'; '32', '1000'; '33', '1000'; '34', '1000'; '35', '1000'; '36', '1000'; '37', '1000'; '38', '1000'; '39', '1000'; '40', '1000'; '41', '1000'; '42', '1000'; '43', '1000'; '44', '1000'; '45', '1000'; '46', '1000'; '47', '1000'; '48', '1000'; '49', '1000'; '50', '1000'; '51', '1000'; '52', '1000'; '53', '1000'; '54', '1000'; '55', '1000'; '56', '1000'; '57', '1000'; '58', '1000'; '59', '1000'; '60', '1000'; '61', '1000'; '62', '1000'; '63', '1000'; '64', '1000' }  Buses_Isc={ '1', '1000'; '2', '1000'; '3', '1000'; '4', '1000'; '5', '1000'; '6', '1000'; '7', '1000'; '8', '1000'; '9', '1000'; '10', '1000'; '11', '1000'; '12', '1000'; '13', '1000'; '14', '1000'; '15', '1000'; '16', '1000'; '17', '1000'; '18', '1000'; '19', '1000'; '20', '1000'; '21', '1000'; '22', '1000'; '23', '1000'; '24', '1000'; '25', '1000'; '26', '1000'; '27', '1000'; '28', '1000'; '29', '1000'; '30', '1000'; '31', '1000'; '32', '1000'; '33', '1000'; '34', '1000'; '35', '1000'; '36', '1000'; '37', '1000'; '38', '1000'; '39', '1000'; '40', '1000'; '41', '1000'; '42', '1000'; '43', '1000'; '44', '1000'; '45', '1000'; '46', '1000'; '47', '1000'; '48', '1000'; '49', '1000'; '50', '1000'; '51', '1000'; '52', '1000'; '53', '1000'; '54', '1000'; '55', '1000'; '56', '1000'; '57', '1000'; '58', '1000'; '59', '1000'; '60', '1000'; '61', '1000'; '62', '1000'; '63', '1000'; '64', '1000'; '65', '1000' }
      settings: SourceProductName=ABB UPPAAL Library
  Source_9 : ABB_UPPAAL_Library/Source_1  MyInitialization=0  Source_ID=9  Lines_Isc={ '1', '1000'; '2', '1000'; '3', '1000'; '4', '1000'; '5', '1000'; '6', '1000'; '7', '1000'; '8', '1000'; '9', '1000'; '10', '1000'; '11', '1000'; '12', '1000'; '13', '1000'; '14', '1000'; '15', '1000'; '16', '1000'; '17', '1000'; '18', '1000'; '19', '1000'; '20', '1000'; '21', '1000'; '22', '1000'; '23', '1000'; '24', '1000'; '25', '1000'; '26', '1000'; '27', '1000'; '28', '1000'; '29', '1000'; '30', '1000'; '31', '1000'; '32', '1000'; '33', '1000'; '34', '1000'; '35', '1000'; '36', '1000'; '37', '1000'; '38', '1000'; '39', '1000'; '40', '1000'; '41', '1000'; '42', '1000'; '43', '1000'; '44', '1000'; '45', '1000'; '46', '1000'; '47', '1000'; '48', '1000'; '49', '1000'; '50', '1000'; '51', '1000'; '52', '1000'; '53', '1000'; '54', '1000'; '55', '1000'; '56', '1000'; '57', '1000'; '58', '1000'; '59', '1000'; '60', '1000'; '61', '1000'; '62', '1000'; '63', '1000'; '64', '1000' }  Buses_Isc={ '1', '1000'; '2', '1000'; '3', '1000'; '4', '1000'; '5', '1000'; '6', '1000'; '7', '1000'; '8', '1000'; '9', '1000'; '10', '1000'; '11', '1000'; '12', '1000'; '13', '1000'; '14', '1000'; '15', '1000'; '16', '1000'; '17', '1000'; '18', '1000'; '19', '1000'; '20', '1000'; '21', '1000'; '22', '1000'; '23', '1000'; '24', '1000'; '25', '1000'; '26', '1000'; '27', '1000'; '28', '1000'; '29', '1000'; '30', '1000'; '31', '1000'; '32', '1000'; '33', '1000'; '34', '1000'; '35', '1000'; '36', '1000'; '37', '1000'; '38', '1000'; '39', '1000'; '40', '1000'; '41', '1000'; '42', '1000'; '43', '1000'; '44', '1000'; '45', '1000'; '46', '1000'; '47', '1000'; '48', '1000'; '49', '1000'; '50', '1000'; '51', '1000'; '52', '1000'; '53', '1000'; '54', '1000'; '55', '1000'; '56', '1000'; '57', '1000'; '58', '1000'; '59', '1000'; '60', '1000'; '61', '1000'; '62', '1000'; '63', '1000'; '64', '1000'; '65', '1000' }
      settings: SourceProductName=ABB UPPAAL Library
  wires:
  Bus_8/1(y) -> Load_3/1
  Line_13/1 -> Bus_14/1(u)
  Line_7/1 -> Bus_8/1(u)
  Bus_9/1(y) -> Line_8/1
  Bus_4/1(y) -> Line_9/1, CB_4/1
  Bus_10/1(y) -> Line_15/1, CB_10/1
  Bus_1/1(y) -> Line_1/1
  Bus_13/1(y) -> CB_14/1, CB_13/1
  Bus_2/1(y) -> Line_2/1
  CB_15/1 -> Bus_21/1(data)
  Line_5/1 -> Bus_6/1(u)
  Line_6/1 -> Bus_7/1(u)
  CB_2/1 -> Bus_4/2(u)
  Bus_12/1(y) -> Load_4/1
  Source_1/1 -> Bus_1/1(u)
  CB_8/1 -> Bus_10/2(u)
  Bus_5/1(y) -> CB_7/1, CB_6/1, CB_5/1
  CB_5/1 -> Line_5/1
  CB_7/1 -> Line_7/1
  Line_3/1 -> CB_3/1
  CB_6/1 -> Line_6/1
  Line_17/1 -> Bus_17/1(u)
  Bus_7/1(y) -> Load_2/1
  Line_15/1 -> CB_15/1
  Line_10/1 -> Bus_11/1(u)
  Line_2/1 -> CB_2/1
  CB_3/1 -> Bus_4/1(data)
  Line_12/1 -> Bus_13/1(u)
  Bus_20/1(y) -> Load_9/1
  Source_16/1 -> Bus_16/1(u)
  Line_11/1 -> Bus_12/1(u)
  Line_8/1 -> CB_8/1
  CB_1/1 -> Bus_3/1(u)
  CB_18/1 -> Line_18/1
  CB_13/1 -> Line_13/1
  CB_9/1 -> Bus_10/1(data)
  Bus_14/1(y) -> Load_5/1
  CB_12/1 -> Line_12/1
  Line_1/1 -> CB_1/1
  CB_14/1 -> Line_14/1
  CB_4/1 -> Line_4/1
  CB_11/1 -> Line_11/1
  Line_16/1 -> CB_16/1
  Source_9/1 -> Bus_9/1(u)
  Bus_15/1(y) -> Load_6/1
  Line_20/1 -> Bus_20/1(u)
  Bus_6/1(y) -> Load_1/1
  Line_14/1 -> Bus_15/1(u)
  Bus_3/1(y) -> Line_3/1
  Bus_11/1(y) -> CB_11/1, CB_12/1
  Line_4/1 -> Bus_5/1(u)
  Source_2/1 -> Bus_2/1(u)
  CB_10/1 -> Line_10/1
  Bus_19/1(y) -> Load_8/1
  Bus_16/1(y) -> Line_16/1
  Line_9/1 -> CB_9/1
  CB_16/1 -> Bus_21/2(u)
  Bus_21/1(y) -> Line_22/1, CB_17/1
  CB_19/1 -> Line_19/1
  Bus_18/1(y) -> Load_7/1
  Bus_17/1(y) -> CB_20/1, CB_19/1, CB_18/1
  Line_19/1 -> Bus_19/1(u)
  CB_20/1 -> Line_20/1
  Line_18/1 -> Bus_18/1(u)
  CB_17/1 -> Line_17/1
  Source_22/1 -> Bus_22/1(u)
  Bus_22/1(y) -> Line_21/1
  Line_21/1 -> CB_21/1
  Line_22/1 -> CB_22/1
  CB_21/1 -> Bus_23/2(u)
  Bus_23/1(y) -> CB_31/1, Line_30/1
  Bus_25/1(y) -> CB_24/1, CB_25/1
  Bus_31/1(y) -> Line_29/1
  Line_26/1 -> Bus_28/1(u)
  CB_29/1 -> Bus_24/2(u)
  Line_27/1 -> Bus_29/1(u)
  CB_23/1 -> Line_23/1
  CB_27/1 -> Line_27/1
  Bus_26/1(y) -> Load_10/1
  Line_25/1 -> Bus_27/1(u)
  Line_24/1 -> Bus_26/1(u)
  CB_25/1 -> Line_25/1
  Line_28/1 -> CB_28/1
  CB_30/1 -> Bus_24/1(data)
  CB_24/1 -> Line_24/1
  Line_30/1 -> CB_30/1
  CB_26/1 -> Line_26/1
  Bus_24/1(y) -> Line_28/1, CB_23/1
  Bus_28/1(y) -> Load_11/1
  Line_29/1 -> CB_29/1
  Source_31/1 -> Bus_31/1(u)
  Line_23/1 -> Bus_25/1(u)
  Bus_27/1(y) -> CB_27/1, CB_26/1
  Bus_29/1(y) -> Load_12/1
  CB_31/1 -> Line_31/1
  Line_31/1 -> Bus_30/1(u)
  Bus_30/1(y) -> Load_13/1
  Bus_34/1(y) -> Load_14/1
  Line_38/1 -> CB_38/1
  Bus_37/1(y) -> Load_16/1
  Bus_36/1(y) -> Load_15/1
  CB_32/1 -> Line_32/1
  Line_36/1 -> Bus_37/1(u)
  Line_33/1 -> Bus_34/1(u)
  Bus_32/1(y) -> Line_37/1, CB_32/1
  Line_32/1 -> Bus_33/1(u)
  CB_35/1 -> Line_35/1
  Bus_33/1(y) -> CB_33/1, CB_34/1
  Bus_35/1(y) -> CB_36/1, CB_35/1
  CB_38/1 -> Bus_32/2(u)
  Line_37/1 -> CB_37/1
  Source_38/1 -> Bus_38/1(u)
  Line_34/1 -> Bus_35/1(u)
  CB_33/1 -> Line_33/1
  Bus_38/1(y) -> Line_38/1
  CB_34/1 -> Line_34/1
  CB_28/1 -> Bus_32/1(data)
  Line_35/1 -> Bus_36/1(u)
  CB_36/1 -> Line_36/1
  Bus_41/1(y) -> Load_17/1
  Line_45/1 -> CB_45/1
  Bus_44/1(y) -> Load_19/1
  Bus_43/1(y) -> Load_18/1
  CB_39/1 -> Line_39/1
  Line_43/1 -> Bus_44/1(u)
  Line_40/1 -> Bus_41/1(u)
  Bus_39/1(y) -> Line_44/1, CB_39/1
  Line_39/1 -> Bus_40/1(u)
  CB_42/1 -> Line_42/1
  Bus_40/1(y) -> CB_40/1, CB_41/1
  Bus_42/1(y) -> CB_43/1, CB_42/1
  CB_45/1 -> Bus_39/2(u)
  Line_44/1 -> CB_44/1
  Source_45/1 -> Bus_45/1(u)
  Line_41/1 -> Bus_42/1(u)
  CB_40/1 -> Line_40/1
  Bus_45/1(y) -> Line_45/1
  CB_41/1 -> Line_41/1
  CB_37/1 -> Bus_39/1(data)
  Line_42/1 -> Bus_43/1(u)
  CB_43/1 -> Line_43/1
  Line_52/1 -> CB_52/1
  Bus_46/1(y) -> Line_51/1, CB_46/1
  CB_52/1 -> Bus_46/2(u)
  Line_51/1 -> CB_51/1
  Source_52/1 -> Bus_52/1(u)
  Bus_52/1(y) -> Line_52/1
  CB_44/1 -> Bus_46/1(data)
  CB_47/1 -> Line_47/1
  CB_49/1 -> Line_49/1
  Line_49/1 -> Bus_50/1(u)
  Bus_50/1(y) -> Load_22/1
  Bus_48/1(y) -> Load_20/1
  Bus_47/1(y) -> CB_49/1, CB_48/1, CB_47/1
  Line_47/1 -> Bus_48/1(u)
  Bus_49/1(y) -> Load_21/1
  CB_48/1 -> Line_48/1
  CB_46/1 -> Line_46/1
  Line_48/1 -> Bus_49/1(u)
  Line_46/1 -> Bus_47/1(u)
  Bus_53/1(y) -> Line_50/1
  Line_50/1 -> CB_50/1
  Source_53/1 -> Bus_53/1(u)
  CB_50/1 -> Bus_51/2(u)
  CB_51/1 -> Bus_51/1(data)
  CB_53/1 -> Line_53/1
  Line_55/1 -> Bus_56/1(u)
  CB_54/1 -> Line_54/1
  Line_54/1 -> Bus_55/1(u)
  Line_56/1 -> Bus_57/1(u)
  CB_56/1 -> Line_56/1
  Bus_55/1(y) -> Load_23/1
  CB_55/1 -> Line_55/1
  Bus_57/1(y) -> Load_25/1
  Bus_54/1(y) -> CB_56/1, CB_55/1, CB_54/1
  Line_53/1 -> Bus_54/1(u)
  Bus_56/1(y) -> Load_24/1
  Line_59/1 -> Bus_60/1(u)
  Line_57/1 -> Bus_58/1(u)
  Bus_58/1(y) -> CB_58/1, CB_59/1
  CB_58/1 -> Line_58/1
  Bus_60/1(y) -> CB_61/1, CB_60/1
  CB_59/1 -> Line_59/1
  Line_58/1 -> Bus_59/1(u)
  CB_61/1 -> Line_61/1
  Line_60/1 -> Bus_61/1(u)
  CB_60/1 -> Line_60/1
  Line_61/1 -> Bus_62/1(u)
  CB_57/1 -> Line_57/1
  Bus_59/1(y) -> Load_26/1
  Bus_61/1(y) -> Load_27/1
  Bus_62/1(y) -> Load_28/1
  Line_64/1 -> Bus_65/1(u)
  Line_62/1 -> Bus_63/1(u)
  Bus_63/1(y) -> CB_64/1, CB_63/1
  CB_63/1 -> Line_63/1
  Bus_65/1(y) -> Load_30/1
  CB_64/1 -> Line_64/1
  Line_63/1 -> Bus_64/1(u)
  CB_62/1 -> Line_62/1
  Bus_64/1(y) -> Load_29/1
  Bus_51/1(y) -> CB_62/1, CB_57/1, CB_53/1
  CB_22/1 -> Bus_23/1(data)
